simulink model "model"  (R2014a)
(part 2 of 2)

      | %<Vbase>V
      | %<VLF>pu
      | %<angleLF>deg.
      | %<Name>
  bus125 : powerlib/Measurements/Load Flow Bus  LConnTagsString=a  ID=bus125  Vbase=110000  Vref=1  Vangle=0  VLF=1  angleLF=0
      settings: AttributesFormatString=|
      | %<ID>
      | %<Vbase>V
      | %<VLF>pu
      | %<angleLF>deg.
      | %<Name>
  bus126 : powerlib/Measurements/Load Flow Bus  LConnTagsString=a  ID=bus126  Vbase=110000  Vref=1  Vangle=0  VLF=1  angleLF=0
      settings: AttributesFormatString=|
      | %<ID>
      | %<Vbase>V
      | %<VLF>pu
      | %<angleLF>deg.
      | %<Name>
  bus127 : powerlib/Measurements/Load Flow Bus  LConnTagsString=a  ID=bus127  Vbase=110000  Vref=1  Vangle=0  VLF=1  angleLF=0
      settings: AttributesFormatString=|
      | %<ID>
      | %<Vbase>V
      | %<VLF>pu
      | %<angleLF>deg.
      | %<Name>
  bus128 : powerlib/Measurements/Load Flow Bus  LConnTagsString=a  ID=bus128  Vbase=110000  Vref=1  Vangle=0  VLF=1  angleLF=0
      settings: AttributesFormatString=|
      | %<ID>
      | %<Vbase>V
      | %<VLF>pu
      | %<angleLF>deg.
      | %<Name>
  bus129 : powerlib/Measurements/Load Flow Bus  LConnTagsString=a  ID=bus129  Vbase=110000  Vref=1  Vangle=0  VLF=1  angleLF=0
      settings: AttributesFormatString=|
      | %<ID>
      | %<Vbase>V
      | %<VLF>pu
      | %<angleLF>deg.
      | %<Name>
  bus13 : powerlib/Measurements/Load Flow Bus  LConnTagsString=a  ID=bus13  Vbase=110000  Vref=1  Vangle=0  VLF=1  angleLF=0
      settings: AttributesFormatString=|
      | %<ID>
      | %<Vbase>V
      | %<VLF>pu
      | %<angleLF>deg.
      | %<Name>
  bus130 : powerlib/Measurements/Load Flow Bus  LConnTagsString=a  ID=bus130  Vbase=110000  Vref=1  Vangle=0  VLF=1  angleLF=0
      settings: AttributesFormatString=|
      | %<ID>
      | %<Vbase>V
      | %<VLF>pu
      | %<angleLF>deg.
      | %<Name>
  bus131 : powerlib/Measurements/Load Flow Bus  LConnTagsString=a  ID=bus131  Vbase=110000  Vref=1  Vangle=0  VLF=1  angleLF=0
      settings: AttributesFormatString=|
      | %<ID>
      | %<Vbase>V
      | %<VLF>pu
      | %<angleLF>deg.
      | %<Name>
  bus132 : powerlib/Measurements/Load Flow Bus  LConnTagsString=a  ID=bus132  Vbase=110000  Vref=1  Vangle=0  VLF=1  angleLF=0
      settings: AttributesFormatString=|
      | %<ID>
      | %<Vbase>V
      | %<VLF>pu
      | %<angleLF>deg.
      | %<Name>
  bus133 : powerlib/Measurements/Load Flow Bus  LConnTagsString=a  ID=bus133  Vbase=110000  Vref=1  Vangle=0  VLF=1  angleLF=0
      settings: AttributesFormatString=|
      | %<ID>
      | %<Vbase>V
      | %<VLF>pu
      | %<angleLF>deg.
      | %<Name>
  bus134 : powerlib/Measurements/Load Flow Bus  LConnTagsString=a  ID=bus134  Vbase=110000  Vref=1  Vangle=0  VLF=1  angleLF=0
      settings: AttributesFormatString=|
      | %<ID>
      | %<Vbase>V
      | %<VLF>pu
      | %<angleLF>deg.
      | %<Name>
  bus135 : powerlib/Measurements/Load Flow Bus  LConnTagsString=a  ID=bus135  Vbase=110000  Vref=1  Vangle=0  VLF=1  angleLF=0
      settings: AttributesFormatString=|
      | %<ID>
      | %<Vbase>V
      | %<VLF>pu
      | %<angleLF>deg.
      | %<Name>
  bus136 : powerlib/Measurements/Load Flow Bus  LConnTagsString=a  ID=bus136  Vbase=220000  Vref=1  Vangle=0  VLF=1  angleLF=0
      settings: AttributesFormatString=|
      | %<ID>
      | %<Vbase>V
      | %<VLF>pu
      | %<angleLF>deg.
      | %<Name>
  bus137 : powerlib/Measurements/Load Flow Bus  LConnTagsString=a  ID=bus137  Vbase=220000  Vref=1  Vangle=0  VLF=1  angleLF=0
      settings: AttributesFormatString=|
      | %<ID>
      | %<Vbase>V
      | %<VLF>pu
      | %<angleLF>deg.
      | %<Name>
  bus138 : powerlib/Measurements/Load Flow Bus  LConnTagsString=a  ID=bus138  Vbase=220000  Vref=1  Vangle=0  VLF=1  angleLF=0
      settings: AttributesFormatString=|
      | %<ID>
      | %<Vbase>V
      | %<VLF>pu
      | %<angleLF>deg.
      | %<Name>
  bus139 : powerlib/Measurements/Load Flow Bus  LConnTagsString=a  ID=bus139  Vbase=220000  Vref=1  Vangle=0  VLF=1  angleLF=0
      settings: AttributesFormatString=|
      | %<ID>
      | %<Vbase>V
      | %<VLF>pu
      | %<angleLF>deg.
      | %<Name>
  bus14 : powerlib/Measurements/Load Flow Bus  LConnTagsString=a  ID=bus14  Vbase=110000  Vref=1  Vangle=0  VLF=1  angleLF=0
      settings: AttributesFormatString=|
      | %<ID>
      | %<Vbase>V
      | %<VLF>pu
      | %<angleLF>deg.
      | %<Name>
  bus140 : powerlib/Measurements/Load Flow Bus  LConnTagsString=a  ID=bus140  Vbase=220000  Vref=1  Vangle=0  VLF=1  angleLF=0
      settings: AttributesFormatString=|
      | %<ID>
      | %<Vbase>V
      | %<VLF>pu
      | %<angleLF>deg.
      | %<Name>
  bus141 : powerlib/Measurements/Load Flow Bus  LConnTagsString=a  ID=bus141  Vbase=220000  Vref=1  Vangle=0  VLF=1  angleLF=0
      settings: AttributesFormatString=|
      | %<ID>
      | %<Vbase>V
      | %<VLF>pu
      | %<angleLF>deg.
      | %<Name>
  bus142 : powerlib/Measurements/Load Flow Bus  LConnTagsString=a  ID=bus142  Vbase=220000  Vref=1  Vangle=0  VLF=1  angleLF=0
      settings: AttributesFormatString=|
      | %<ID>
      | %<Vbase>V
      | %<VLF>pu
      | %<angleLF>deg.
      | %<Name>
  bus143 : powerlib/Measurements/Load Flow Bus  LConnTagsString=a  ID=bus143  Vbase=220000  Vref=1  Vangle=0  VLF=1  angleLF=0
      settings: AttributesFormatString=|
      | %<ID>
      | %<Vbase>V
      | %<VLF>pu
      | %<angleLF>deg.
      | %<Name>
  bus144 : powerlib/Measurements/Load Flow Bus  LConnTagsString=a  ID=bus144  Vbase=220000  Vref=1  Vangle=0  VLF=1  angleLF=0
      settings: AttributesFormatString=|
      | %<ID>
      | %<Vbase>V
      | %<VLF>pu
      | %<angleLF>deg.
      | %<Name>
  bus145 : powerlib/Measurements/Load Flow Bus  LConnTagsString=a  ID=bus145  Vbase=220000  Vref=1  Vangle=0  VLF=1  angleLF=0
      settings: AttributesFormatString=|
      | %<ID>
      | %<Vbase>V
      | %<VLF>pu
      | %<angleLF>deg.
      | %<Name>
  bus146 : powerlib/Measurements/Load Flow Bus  LConnTagsString=a  ID=bus146  Vbase=220000  Vref=1  Vangle=0  VLF=1  angleLF=0
      settings: AttributesFormatString=|
      | %<ID>
      | %<Vbase>V
      | %<VLF>pu
      | %<angleLF>deg.
      | %<Name>
  bus147 : powerlib/Measurements/Load Flow Bus  LConnTagsString=a  ID=bus147  Vbase=220000  Vref=1  Vangle=0  VLF=1  angleLF=0
      settings: AttributesFormatString=|
      | %<ID>
      | %<Vbase>V
      | %<VLF>pu
      | %<angleLF>deg.
      | %<Name>
  bus148 : powerlib/Measurements/Load Flow Bus  LConnTagsString=a  ID=bus148  Vbase=220000  Vref=1  Vangle=0  VLF=1  angleLF=0
      settings: AttributesFormatString=|
      | %<ID>
      | %<Vbase>V
      | %<VLF>pu
      | %<angleLF>deg.
      | %<Name>
  bus149 : powerlib/Measurements/Load Flow Bus  LConnTagsString=a  ID=bus149  Vbase=220000  Vref=1  Vangle=0  VLF=1  angleLF=0
      settings: AttributesFormatString=|
      | %<ID>
      | %<Vbase>V
      | %<VLF>pu
      | %<angleLF>deg.
      | %<Name>
  bus15 : powerlib/Measurements/Load Flow Bus  LConnTagsString=a  ID=bus15  Vbase=110000  Vref=1  Vangle=0  VLF=1  angleLF=0
      settings: AttributesFormatString=|
      | %<ID>
      | %<Vbase>V
      | %<VLF>pu
      | %<angleLF>deg.
      | %<Name>
  bus150 : powerlib/Measurements/Load Flow Bus  LConnTagsString=a  ID=bus150  Vbase=220000  Vref=1  Vangle=0  VLF=1  angleLF=0
      settings: AttributesFormatString=|
      | %<ID>
      | %<Vbase>V
      | %<VLF>pu
      | %<angleLF>deg.
      | %<Name>
  bus151 : powerlib/Measurements/Load Flow Bus  LConnTagsString=a  ID=bus151  Vbase=220000  Vref=1  Vangle=0  VLF=1  angleLF=0
      settings: AttributesFormatString=|
      | %<ID>
      | %<Vbase>V
      | %<VLF>pu
      | %<angleLF>deg.
      | %<Name>
  bus152 : powerlib/Measurements/Load Flow Bus  LConnTagsString=a  ID=bus152  Vbase=220000  Vref=1  Vangle=0  VLF=1  angleLF=0
      settings: AttributesFormatString=|
      | %<ID>
      | %<Vbase>V
      | %<VLF>pu
      | %<angleLF>deg.
      | %<Name>
  bus153 : powerlib/Measurements/Load Flow Bus  LConnTagsString=a  ID=bus153  Vbase=220000  Vref=1  Vangle=0  VLF=1  angleLF=0
      settings: AttributesFormatString=|
      | %<ID>
      | %<Vbase>V
      | %<VLF>pu
      | %<angleLF>deg.
      | %<Name>
  bus154 : powerlib/Measurements/Load Flow Bus  LConnTagsString=a  ID=bus154  Vbase=220000  Vref=1  Vangle=0  VLF=1  angleLF=0
      settings: AttributesFormatString=|
      | %<ID>
      | %<Vbase>V
      | %<VLF>pu
      | %<angleLF>deg.
      | %<Name>
  bus155 : powerlib/Measurements/Load Flow Bus  LConnTagsString=a  ID=bus155  Vbase=220000  Vref=1  Vangle=0  VLF=1  angleLF=0
      settings: AttributesFormatString=|
      | %<ID>
      | %<Vbase>V
      | %<VLF>pu
      | %<angleLF>deg.
      | %<Name>
  bus156 : powerlib/Measurements/Load Flow Bus  LConnTagsString=a  ID=bus156  Vbase=220000  Vref=1  Vangle=0  VLF=1  angleLF=0
      settings: AttributesFormatString=|
      | %<ID>
      | %<Vbase>V
      | %<VLF>pu
      | %<angleLF>deg.
      | %<Name>
  bus157 : powerlib/Measurements/Load Flow Bus  LConnTagsString=a  ID=bus157  Vbase=220000  Vref=1  Vangle=0  VLF=1  angleLF=0
      settings: AttributesFormatString=|
      | %<ID>
      | %<Vbase>V
      | %<VLF>pu
      | %<angleLF>deg.
      | %<Name>
  bus158 : powerlib/Measurements/Load Flow Bus  LConnTagsString=a  ID=bus158  Vbase=220000  Vref=1  Vangle=0  VLF=1  angleLF=0
      settings: AttributesFormatString=|
      | %<ID>
      | %<Vbase>V
      | %<VLF>pu
      | %<angleLF>deg.
      | %<Name>
  bus159 : powerlib/Measurements/Load Flow Bus  LConnTagsString=a  ID=bus159  Vbase=220000  Vref=1  Vangle=0  VLF=1  angleLF=0
      settings: AttributesFormatString=|
      | %<ID>
      | %<Vbase>V
      | %<VLF>pu
      | %<angleLF>deg.
      | %<Name>
  bus16 : powerlib/Measurements/Load Flow Bus  LConnTagsString=a  ID=bus16  Vbase=110000  Vref=1  Vangle=0  VLF=1  angleLF=0
      settings: AttributesFormatString=|
      | %<ID>
      | %<Vbase>V
      | %<VLF>pu
      | %<angleLF>deg.
      | %<Name>
  bus160 : powerlib/Measurements/Load Flow Bus  LConnTagsString=a  ID=bus160  Vbase=220000  Vref=1  Vangle=0  VLF=1  angleLF=0
      settings: AttributesFormatString=|
      | %<ID>
      | %<Vbase>V
      | %<VLF>pu
      | %<angleLF>deg.
      | %<Name>
  bus161 : powerlib/Measurements/Load Flow Bus  LConnTagsString=a  ID=bus161  Vbase=220000  Vref=1  Vangle=0  VLF=1  angleLF=0
      settings: AttributesFormatString=|
      | %<ID>
      | %<Vbase>V
      | %<VLF>pu
      | %<angleLF>deg.
      | %<Name>
  bus162 : powerlib/Measurements/Load Flow Bus  LConnTagsString=a  ID=bus162  Vbase=220000  Vref=1  Vangle=0  VLF=1  angleLF=0
      settings: AttributesFormatString=|
      | %<ID>
      | %<Vbase>V
      | %<VLF>pu
      | %<angleLF>deg.
      | %<Name>
  bus163 : powerlib/Measurements/Load Flow Bus  LConnTagsString=a  ID=bus163  Vbase=220000  Vref=1  Vangle=0  VLF=1  angleLF=0
      settings: AttributesFormatString=|
      | %<ID>
      | %<Vbase>V
      | %<VLF>pu
      | %<angleLF>deg.
      | %<Name>
  bus164 : powerlib/Measurements/Load Flow Bus  LConnTagsString=a  ID=bus164  Vbase=220000  Vref=1  Vangle=0  VLF=1  angleLF=0
      settings: AttributesFormatString=|
      | %<ID>
      | %<Vbase>V
      | %<VLF>pu
      | %<angleLF>deg.
      | %<Name>
  bus165 : powerlib/Measurements/Load Flow Bus  LConnTagsString=a  ID=bus165  Vbase=220000  Vref=1  Vangle=0  VLF=1  angleLF=0
      settings: AttributesFormatString=|
      | %<ID>
      | %<Vbase>V
      | %<VLF>pu
      | %<angleLF>deg.
      | %<Name>
  bus166 : powerlib/Measurements/Load Flow Bus  LConnTagsString=a  ID=bus166  Vbase=220000  Vref=1  Vangle=0  VLF=1  angleLF=0
      settings: AttributesFormatString=|
      | %<ID>
      | %<Vbase>V
      | %<VLF>pu
      | %<angleLF>deg.
      | %<Name>
  bus167 : powerlib/Measurements/Load Flow Bus  LConnTagsString=a  ID=bus167  Vbase=220000  Vref=1  Vangle=0  VLF=1  angleLF=0
      settings: AttributesFormatString=|
      | %<ID>
      | %<Vbase>V
      | %<VLF>pu
      | %<angleLF>deg.
      | %<Name>
  bus168 : powerlib/Measurements/Load Flow Bus  LConnTagsString=a  ID=bus168  Vbase=220000  Vref=1  Vangle=0  VLF=1  angleLF=0
      settings: AttributesFormatString=|
      | %<ID>
      | %<Vbase>V
      | %<VLF>pu
      | %<angleLF>deg.
      | %<Name>
  bus169 : powerlib/Measurements/Load Flow Bus  LConnTagsString=a  ID=bus169  Vbase=220000  Vref=1  Vangle=0  VLF=1  angleLF=0
      settings: AttributesFormatString=|
      | %<ID>
      | %<Vbase>V
      | %<VLF>pu
      | %<angleLF>deg.
      | %<Name>
  bus17 : powerlib/Measurements/Load Flow Bus  LConnTagsString=a  ID=bus17  Vbase=110000  Vref=1  Vangle=0  VLF=1  angleLF=0
      settings: AttributesFormatString=|
      | %<ID>
      | %<Vbase>V
      | %<VLF>pu
      | %<angleLF>deg.
      | %<Name>
  bus170 : powerlib/Measurements/Load Flow Bus  LConnTagsString=a  ID=bus170  Vbase=220000  Vref=1  Vangle=0  VLF=1  angleLF=0
      settings: AttributesFormatString=|
      | %<ID>
      | %<Vbase>V
      | %<VLF>pu
      | %<angleLF>deg.
      | %<Name>
  bus171 : powerlib/Measurements/Load Flow Bus  LConnTagsString=a  ID=bus171  Vbase=220000  Vref=1  Vangle=0  VLF=1  angleLF=0
      settings: AttributesFormatString=|
      | %<ID>
      | %<Vbase>V
      | %<VLF>pu
      | %<angleLF>deg.
      | %<Name>
  bus172 : powerlib/Measurements/Load Flow Bus  LConnTagsString=a  ID=bus172  Vbase=220000  Vref=1  Vangle=0  VLF=1  angleLF=0
      settings: AttributesFormatString=|
      | %<ID>
      | %<Vbase>V
      | %<VLF>pu
      | %<angleLF>deg.
      | %<Name>
  bus173 : powerlib/Measurements/Load Flow Bus  LConnTagsString=a  ID=bus173  Vbase=220000  Vref=1  Vangle=0  VLF=1  angleLF=0
      settings: AttributesFormatString=|
      | %<ID>
      | %<Vbase>V
      | %<VLF>pu
      | %<angleLF>deg.
      | %<Name>
  bus174 : powerlib/Measurements/Load Flow Bus  LConnTagsString=a  ID=bus174  Vbase=220000  Vref=1  Vangle=0  VLF=1  angleLF=0
      settings: AttributesFormatString=|
      | %<ID>
      | %<Vbase>V
      | %<VLF>pu
      | %<angleLF>deg.
      | %<Name>
  bus175 : powerlib/Measurements/Load Flow Bus  LConnTagsString=a  ID=bus175  Vbase=220000  Vref=1  Vangle=0  VLF=1  angleLF=0
      settings: AttributesFormatString=|
      | %<ID>
      | %<Vbase>V
      | %<VLF>pu
      | %<angleLF>deg.
      | %<Name>
  bus176 : powerlib/Measurements/Load Flow Bus  LConnTagsString=a  ID=bus176  Vbase=220000  Vref=1  Vangle=0  VLF=1  angleLF=0
      settings: AttributesFormatString=|
      | %<ID>
      | %<Vbase>V
      | %<VLF>pu
      | %<angleLF>deg.
      | %<Name>
  bus177 : powerlib/Measurements/Load Flow Bus  LConnTagsString=a  ID=bus177  Vbase=220000  Vref=1  Vangle=0  VLF=1  angleLF=0
      settings: AttributesFormatString=|
      | %<ID>
      | %<Vbase>V
      | %<VLF>pu
      | %<angleLF>deg.
      | %<Name>
  bus178 : powerlib/Measurements/Load Flow Bus  LConnTagsString=a  ID=bus178  Vbase=220000  Vref=1  Vangle=0  VLF=1  angleLF=0
      settings: AttributesFormatString=|
      | %<ID>
      | %<Vbase>V
      | %<VLF>pu
      | %<angleLF>deg.
      | %<Name>
  bus179 : powerlib/Measurements/Load Flow Bus  LConnTagsString=a  ID=bus179  Vbase=220000  Vref=1  Vangle=0  VLF=1  angleLF=0
      settings: AttributesFormatString=|
      | %<ID>
      | %<Vbase>V
      | %<VLF>pu
      | %<angleLF>deg.
      | %<Name>
  bus18 : powerlib/Measurements/Load Flow Bus  LConnTagsString=a  ID=bus18  Vbase=110000  Vref=1  Vangle=0  VLF=1  angleLF=0
      settings: AttributesFormatString=|
      | %<ID>
      | %<Vbase>V
      | %<VLF>pu
      | %<angleLF>deg.
      | %<Name>
  bus180 : powerlib/Measurements/Load Flow Bus  LConnTagsString=a  ID=bus180  Vbase=220000  Vref=1  Vangle=0  VLF=1  angleLF=0
      settings: AttributesFormatString=|
      | %<ID>
      | %<Vbase>V
      | %<VLF>pu
      | %<angleLF>deg.
      | %<Name>
  bus181 : powerlib/Measurements/Load Flow Bus  LConnTagsString=a  ID=bus181  Vbase=220000  Vref=1  Vangle=0  VLF=1  angleLF=0
      settings: AttributesFormatString=|
      | %<ID>
      | %<Vbase>V
      | %<VLF>pu
      | %<angleLF>deg.
      | %<Name>
  bus182 : powerlib/Measurements/Load Flow Bus  LConnTagsString=a  ID=bus182  Vbase=220000  Vref=1  Vangle=0  VLF=1  angleLF=0
      settings: AttributesFormatString=|
      | %<ID>
      | %<Vbase>V
      | %<VLF>pu
      | %<angleLF>deg.
      | %<Name>
  bus183 : powerlib/Measurements/Load Flow Bus  LConnTagsString=a  ID=bus183  Vbase=220000  Vref=1  Vangle=0  VLF=1  angleLF=0
      settings: AttributesFormatString=|
      | %<ID>
      | %<Vbase>V
      | %<VLF>pu
      | %<angleLF>deg.
      | %<Name>
  bus184 : powerlib/Measurements/Load Flow Bus  LConnTagsString=a  ID=bus184  Vbase=220000  Vref=1  Vangle=0  VLF=1  angleLF=0
      settings: AttributesFormatString=|
      | %<ID>
      | %<Vbase>V
      | %<VLF>pu
      | %<angleLF>deg.
      | %<Name>
  bus185 : powerlib/Measurements/Load Flow Bus  LConnTagsString=a  ID=bus185  Vbase=220000  Vref=1  Vangle=0  VLF=1  angleLF=0
      settings: AttributesFormatString=|
      | %<ID>
      | %<Vbase>V
      | %<VLF>pu
      | %<angleLF>deg.
      | %<Name>
  bus186 : powerlib/Measurements/Load Flow Bus  LConnTagsString=a  ID=bus186  Vbase=220000  Vref=1  Vangle=0  VLF=1  angleLF=0
      settings: AttributesFormatString=|
      | %<ID>
      | %<Vbase>V
      | %<VLF>pu
      | %<angleLF>deg.
      | %<Name>
  bus187 : powerlib/Measurements/Load Flow Bus  LConnTagsString=a  ID=bus187  Vbase=220000  Vref=1  Vangle=0  VLF=1  angleLF=0
      settings: AttributesFormatString=|
      | %<ID>
      | %<Vbase>V
      | %<VLF>pu
      | %<angleLF>deg.
      | %<Name>
  bus188 : powerlib/Measurements/Load Flow Bus  LConnTagsString=a  ID=bus188  Vbase=220000  Vref=1  Vangle=0  VLF=1  angleLF=0
      settings: AttributesFormatString=|
      | %<ID>
      | %<Vbase>V
      | %<VLF>pu
      | %<angleLF>deg.
      | %<Name>
  bus189 : powerlib/Measurements/Load Flow Bus  LConnTagsString=a  ID=bus189  Vbase=220000  Vref=1  Vangle=0  VLF=1  angleLF=0
      settings: AttributesFormatString=|
      | %<ID>
      | %<Vbase>V
      | %<VLF>pu
      | %<angleLF>deg.
      | %<Name>
  bus19 : powerlib/Measurements/Load Flow Bus  LConnTagsString=a  ID=bus19  Vbase=110000  Vref=1  Vangle=0  VLF=1  angleLF=0
      settings: AttributesFormatString=|
      | %<ID>
      | %<Vbase>V
      | %<VLF>pu
      | %<angleLF>deg.
      | %<Name>
  bus190 : powerlib/Measurements/Load Flow Bus  LConnTagsString=a  ID=bus190  Vbase=220000  Vref=1  Vangle=0  VLF=1  angleLF=0
      settings: AttributesFormatString=|
      | %<ID>
      | %<Vbase>V
      | %<VLF>pu
      | %<angleLF>deg.
      | %<Name>
  bus191 : powerlib/Measurements/Load Flow Bus  LConnTagsString=a  ID=bus191  Vbase=220000  Vref=1  Vangle=0  VLF=1  angleLF=0
      settings: AttributesFormatString=|
      | %<ID>
      | %<Vbase>V
      | %<VLF>pu
      | %<angleLF>deg.
      | %<Name>
  bus192 : powerlib/Measurements/Load Flow Bus  LConnTagsString=a  ID=bus192  Vbase=220000  Vref=1  Vangle=0  VLF=1  angleLF=0
      settings: AttributesFormatString=|
      | %<ID>
      | %<Vbase>V
      | %<VLF>pu
      | %<angleLF>deg.
      | %<Name>
  bus193 : powerlib/Measurements/Load Flow Bus  LConnTagsString=a  ID=bus193  Vbase=220000  Vref=1  Vangle=0  VLF=1  angleLF=0
      settings: AttributesFormatString=|
      | %<ID>
      | %<Vbase>V
      | %<VLF>pu
      | %<angleLF>deg.
      | %<Name>
  bus194 : powerlib/Measurements/Load Flow Bus  LConnTagsString=a  ID=bus194  Vbase=220000  Vref=1  Vangle=0  VLF=1  angleLF=0
      settings: AttributesFormatString=|
      | %<ID>
      | %<Vbase>V
      | %<VLF>pu
      | %<angleLF>deg.
      | %<Name>
  bus195 : powerlib/Measurements/Load Flow Bus  LConnTagsString=a  ID=bus195  Vbase=220000  Vref=1  Vangle=0  VLF=1  angleLF=0
      settings: AttributesFormatString=|
      | %<ID>
      | %<Vbase>V
      | %<VLF>pu
      | %<angleLF>deg.
      | %<Name>
  bus196 : powerlib/Measurements/Load Flow Bus  LConnTagsString=a  ID=bus196  Vbase=220000  Vref=1  Vangle=0  VLF=1  angleLF=0
      settings: AttributesFormatString=|
      | %<ID>
      | %<Vbase>V
      | %<VLF>pu
      | %<angleLF>deg.
      | %<Name>
  bus197 : powerlib/Measurements/Load Flow Bus  LConnTagsString=a  ID=bus197  Vbase=220000  Vref=1  Vangle=0  VLF=1  angleLF=0
      settings: AttributesFormatString=|
      | %<ID>
      | %<Vbase>V
      | %<VLF>pu
      | %<angleLF>deg.
      | %<Name>
  bus198 : powerlib/Measurements/Load Flow Bus  LConnTagsString=a  ID=bus198  Vbase=220000  Vref=1  Vangle=0  VLF=1  angleLF=0
      settings: AttributesFormatString=|
      | %<ID>
      | %<Vbase>V
      | %<VLF>pu
      | %<angleLF>deg.
      | %<Name>
  bus199 : powerlib/Measurements/Load Flow Bus  LConnTagsString=a  ID=bus199  Vbase=220000  Vref=1  Vangle=0  VLF=1  angleLF=0
      settings: AttributesFormatString=|
      | %<ID>
      | %<Vbase>V
      | %<VLF>pu
      | %<angleLF>deg.
      | %<Name>
  bus2 : powerlib/Measurements/Load Flow Bus  LConnTagsString=a  ID=bus2  Vbase=110000  Vref=1  Vangle=0  VLF=1  angleLF=0
      settings: AttributesFormatString=|
      | %<ID>
      | %<Vbase>V
      | %<VLF>pu
      | %<angleLF>deg.
      | %<Name>
  bus20 : powerlib/Measurements/Load Flow Bus  LConnTagsString=a  ID=bus20  Vbase=110000  Vref=1  Vangle=0  VLF=1  angleLF=0
      settings: AttributesFormatString=|
      | %<ID>
      | %<Vbase>V
      | %<VLF>pu
      | %<angleLF>deg.
      | %<Name>
  bus200 : powerlib/Measurements/Load Flow Bus  LConnTagsString=a  ID=bus200  Vbase=220000  Vref=1  Vangle=0  VLF=1  angleLF=0
      settings: AttributesFormatString=|
      | %<ID>
      | %<Vbase>V
      | %<VLF>pu
      | %<angleLF>deg.
      | %<Name>
  bus201 : powerlib/Measurements/Load Flow Bus  LConnTagsString=a  ID=bus201  Vbase=220000  Vref=1  Vangle=0  VLF=1  angleLF=0
      settings: AttributesFormatString=|
      | %<ID>
      | %<Vbase>V
      | %<VLF>pu
      | %<angleLF>deg.
      | %<Name>
  bus202 : powerlib/Measurements/Load Flow Bus  LConnTagsString=a  ID=bus202  Vbase=220000  Vref=1  Vangle=0  VLF=1  angleLF=0
      settings: AttributesFormatString=|
      | %<ID>
      | %<Vbase>V
      | %<VLF>pu
      | %<angleLF>deg.
      | %<Name>
  bus203 : powerlib/Measurements/Load Flow Bus  LConnTagsString=a  ID=bus203  Vbase=220000  Vref=1  Vangle=0  VLF=1  angleLF=0
      settings: AttributesFormatString=|
      | %<ID>
      | %<Vbase>V
      | %<VLF>pu
      | %<angleLF>deg.
      | %<Name>
  bus204 : powerlib/Measurements/Load Flow Bus  LConnTagsString=a  ID=bus204  Vbase=220000  Vref=1  Vangle=0  VLF=1  angleLF=0
      settings: AttributesFormatString=|
      | %<ID>
      | %<Vbase>V
      | %<VLF>pu
      | %<angleLF>deg.
      | %<Name>
  bus205 : powerlib/Measurements/Load Flow Bus  LConnTagsString=a  ID=bus205  Vbase=220000  Vref=1  Vangle=0  VLF=1  angleLF=0
      settings: AttributesFormatString=|
      | %<ID>
      | %<Vbase>V
      | %<VLF>pu
      | %<angleLF>deg.
      | %<Name>
  bus206 : powerlib/Measurements/Load Flow Bus  LConnTagsString=a  ID=bus206  Vbase=220000  Vref=1  Vangle=0  VLF=1  angleLF=0
      settings: AttributesFormatString=|
      | %<ID>
      | %<Vbase>V
      | %<VLF>pu
      | %<angleLF>deg.
      | %<Name>
  bus207 : powerlib/Measurements/Load Flow Bus  LConnTagsString=a  ID=bus207  Vbase=220000  Vref=1  Vangle=0  VLF=1  angleLF=0
      settings: AttributesFormatString=|
      | %<ID>
      | %<Vbase>V
      | %<VLF>pu
      | %<angleLF>deg.
      | %<Name>
  bus208 : powerlib/Measurements/Load Flow Bus  LConnTagsString=a  ID=bus208  Vbase=220000  Vref=1  Vangle=0  VLF=1  angleLF=0
      settings: AttributesFormatString=|
      | %<ID>
      | %<Vbase>V
      | %<VLF>pu
      | %<angleLF>deg.
      | %<Name>
  bus209 : powerlib/Measurements/Load Flow Bus  LConnTagsString=a  ID=bus209  Vbase=220000  Vref=1  Vangle=0  VLF=1  angleLF=0
      settings: AttributesFormatString=|
      | %<ID>
      | %<Vbase>V
      | %<VLF>pu
      | %<angleLF>deg.
      | %<Name>
  bus21 : powerlib/Measurements/Load Flow Bus  LConnTagsString=a  ID=bus21  Vbase=110000  Vref=1  Vangle=0  VLF=1  angleLF=0
      settings: AttributesFormatString=|
      | %<ID>
      | %<Vbase>V
      | %<VLF>pu
      | %<angleLF>deg.
      | %<Name>
  bus210 : powerlib/Measurements/Load Flow Bus  LConnTagsString=a  ID=bus210  Vbase=220000  Vref=1  Vangle=0  VLF=1  angleLF=0
      settings: AttributesFormatString=|
      | %<ID>
      | %<Vbase>V
      | %<VLF>pu
      | %<angleLF>deg.
      | %<Name>
  bus211 : powerlib/Measurements/Load Flow Bus  LConnTagsString=a  ID=bus211  Vbase=220000  Vref=1  Vangle=0  VLF=1  angleLF=0
      settings: AttributesFormatString=|
      | %<ID>
      | %<Vbase>V
      | %<VLF>pu
      | %<angleLF>deg.
      | %<Name>
  bus212 : powerlib/Measurements/Load Flow Bus  LConnTagsString=a  ID=bus212  Vbase=220000  Vref=1  Vangle=0  VLF=1  angleLF=0
      settings: AttributesFormatString=|
      | %<ID>
      | %<Vbase>V
      | %<VLF>pu
      | %<angleLF>deg.
      | %<Name>
  bus213 : powerlib/Measurements/Load Flow Bus  LConnTagsString=a  ID=bus213  Vbase=220000  Vref=1  Vangle=0  VLF=1  angleLF=0
      settings: AttributesFormatString=|
      | %<ID>
      | %<Vbase>V
      | %<VLF>pu
      | %<angleLF>deg.
      | %<Name>
  bus214 : powerlib/Measurements/Load Flow Bus  LConnTagsString=a  ID=bus214  Vbase=220000  Vref=1  Vangle=0  VLF=1  angleLF=0
      settings: AttributesFormatString=|
      | %<ID>
      | %<Vbase>V
      | %<VLF>pu
      | %<angleLF>deg.
      | %<Name>
  bus215 : powerlib/Measurements/Load Flow Bus  LConnTagsString=a  ID=bus215  Vbase=220000  Vref=1  Vangle=0  VLF=1  angleLF=0
      settings: AttributesFormatString=|
      | %<ID>
      | %<Vbase>V
      | %<VLF>pu
      | %<angleLF>deg.
      | %<Name>
  bus216 : powerlib/Measurements/Load Flow Bus  LConnTagsString=a  ID=bus216  Vbase=220000  Vref=1  Vangle=0  VLF=1  angleLF=0
      settings: AttributesFormatString=|
      | %<ID>
      | %<Vbase>V
      | %<VLF>pu
      | %<angleLF>deg.
      | %<Name>
  bus217 : powerlib/Measurements/Load Flow Bus  LConnTagsString=a  ID=bus217  Vbase=220000  Vref=1  Vangle=0  VLF=1  angleLF=0
      settings: AttributesFormatString=|
      | %<ID>
      | %<Vbase>V
      | %<VLF>pu
      | %<angleLF>deg.
      | %<Name>
  bus218 : powerlib/Measurements/Load Flow Bus  LConnTagsString=a  ID=bus218  Vbase=220000  Vref=1  Vangle=0  VLF=1  angleLF=0
      settings: AttributesFormatString=|
      | %<ID>
      | %<Vbase>V
      | %<VLF>pu
      | %<angleLF>deg.
      | %<Name>
  bus219 : powerlib/Measurements/Load Flow Bus  LConnTagsString=a  ID=bus219  Vbase=220000  Vref=1  Vangle=0  VLF=1  angleLF=0
      settings: AttributesFormatString=|
      | %<ID>
      | %<Vbase>V
      | %<VLF>pu
      | %<angleLF>deg.
      | %<Name>
  bus22 : powerlib/Measurements/Load Flow Bus  LConnTagsString=a  ID=bus22  Vbase=110000  Vref=1  Vangle=0  VLF=1  angleLF=0
      settings: AttributesFormatString=|
      | %<ID>
      | %<Vbase>V
      | %<VLF>pu
      | %<angleLF>deg.
      | %<Name>
  bus220 : powerlib/Measurements/Load Flow Bus  LConnTagsString=a  ID=bus220  Vbase=220000  Vref=1  Vangle=0  VLF=1  angleLF=0
      settings: AttributesFormatString=|
      | %<ID>
      | %<Vbase>V
      | %<VLF>pu
      | %<angleLF>deg.
      | %<Name>
  bus221 : powerlib/Measurements/Load Flow Bus  LConnTagsString=a  ID=bus221  Vbase=220000  Vref=1  Vangle=0  VLF=1  angleLF=0
      settings: AttributesFormatString=|
      | %<ID>
      | %<Vbase>V
      | %<VLF>pu
      | %<angleLF>deg.
      | %<Name>
  bus222 : powerlib/Measurements/Load Flow Bus  LConnTagsString=a  ID=bus222  Vbase=220000  Vref=1  Vangle=0  VLF=1  angleLF=0
      settings: AttributesFormatString=|
      | %<ID>
      | %<Vbase>V
      | %<VLF>pu
      | %<angleLF>deg.
      | %<Name>
  bus23 : powerlib/Measurements/Load Flow Bus  LConnTagsString=a  ID=bus23  Vbase=110000  Vref=1  Vangle=0  VLF=1  angleLF=0
      settings: AttributesFormatString=|
      | %<ID>
      | %<Vbase>V
      | %<VLF>pu
      | %<angleLF>deg.
      | %<Name>
  bus24 : powerlib/Measurements/Load Flow Bus  LConnTagsString=a  ID=bus24  Vbase=110000  Vref=1  Vangle=0  VLF=1  angleLF=0
      settings: AttributesFormatString=|
      | %<ID>
      | %<Vbase>V
      | %<VLF>pu
      | %<angleLF>deg.
      | %<Name>
  bus25 : powerlib/Measurements/Load Flow Bus  LConnTagsString=a  ID=bus25  Vbase=220000  Vref=1  Vangle=0  VLF=1  angleLF=0
      settings: AttributesFormatString=|
      | %<ID>
      | %<Vbase>V
      | %<VLF>pu
      | %<angleLF>deg.
      | %<Name>
  bus26 : powerlib/Measurements/Load Flow Bus  LConnTagsString=a  ID=bus26  Vbase=220000  Vref=1  Vangle=0  VLF=1  angleLF=0
      settings: AttributesFormatString=|
      | %<ID>
      | %<Vbase>V
      | %<VLF>pu
      | %<angleLF>deg.
      | %<Name>
  bus27 : powerlib/Measurements/Load Flow Bus  LConnTagsString=a  ID=bus27  Vbase=220000  Vref=1  Vangle=0  VLF=1  angleLF=0
      settings: AttributesFormatString=|
      | %<ID>
      | %<Vbase>V
      | %<VLF>pu
      | %<angleLF>deg.
      | %<Name>
  bus28 : powerlib/Measurements/Load Flow Bus  LConnTagsString=a  ID=bus28  Vbase=220000  Vref=1  Vangle=0  VLF=1  angleLF=0
      settings: AttributesFormatString=|
      | %<ID>
      | %<Vbase>V
      | %<VLF>pu
      | %<angleLF>deg.
      | %<Name>
  bus29 : powerlib/Measurements/Load Flow Bus  LConnTagsString=a  ID=bus29  Vbase=220000  Vref=1  Vangle=0  VLF=1  angleLF=0
      settings: AttributesFormatString=|
      | %<ID>
      | %<Vbase>V
      | %<VLF>pu
      | %<angleLF>deg.
      | %<Name>
  bus3 : powerlib/Measurements/Load Flow Bus  LConnTagsString=a  ID=bus3  Vbase=110000  Vref=1  Vangle=0  VLF=1  angleLF=0
      settings: AttributesFormatString=|
      | %<ID>
      | %<Vbase>V
      | %<VLF>pu
      | %<angleLF>deg.
      | %<Name>
  bus30 : powerlib/Measurements/Load Flow Bus  LConnTagsString=a  ID=bus30  Vbase=220000  Vref=1  Vangle=0  VLF=1  angleLF=0
      settings: AttributesFormatString=|
      | %<ID>
      | %<Vbase>V
      | %<VLF>pu
      | %<angleLF>deg.
      | %<Name>
  bus31 : powerlib/Measurements/Load Flow Bus  LConnTagsString=a  ID=bus31  Vbase=220000  Vref=1  Vangle=0  VLF=1  angleLF=0
      settings: AttributesFormatString=|
      | %<ID>
      | %<Vbase>V
      | %<VLF>pu
      | %<angleLF>deg.
      | %<Name>
  bus32 : powerlib/Measurements/Load Flow Bus  LConnTagsString=a  ID=bus32  Vbase=220000  Vref=1  Vangle=0  VLF=1  angleLF=0
      settings: AttributesFormatString=|
      | %<ID>
      | %<Vbase>V
      | %<VLF>pu
      | %<angleLF>deg.
      | %<Name>
  bus33 : powerlib/Measurements/Load Flow Bus  LConnTagsString=a  ID=bus33  Vbase=220000  Vref=1  Vangle=0  VLF=1  angleLF=0
      settings: AttributesFormatString=|
      | %<ID>
      | %<Vbase>V
      | %<VLF>pu
      | %<angleLF>deg.
      | %<Name>
  bus34 : powerlib/Measurements/Load Flow Bus  LConnTagsString=a  ID=bus34  Vbase=220000  Vref=1  Vangle=0  VLF=1  angleLF=0
      settings: AttributesFormatString=|
      | %<ID>
      | %<Vbase>V
      | %<VLF>pu
      | %<angleLF>deg.
      | %<Name>
  bus35 : powerlib/Measurements/Load Flow Bus  LConnTagsString=a  ID=bus35  Vbase=220000  Vref=1  Vangle=0  VLF=1  angleLF=0
      settings: AttributesFormatString=|
      | %<ID>
      | %<Vbase>V
      | %<VLF>pu
      | %<angleLF>deg.
      | %<Name>
  bus36 : powerlib/Measurements/Load Flow Bus  LConnTagsString=a  ID=bus36  Vbase=220000  Vref=1  Vangle=0  VLF=1  angleLF=0
      settings: AttributesFormatString=|
      | %<ID>
      | %<Vbase>V
      | %<VLF>pu
      | %<angleLF>deg.
      | %<Name>
  bus37 : powerlib/Measurements/Load Flow Bus  LConnTagsString=a  ID=bus37  Vbase=220000  Vref=1  Vangle=0  VLF=1  angleLF=0
      settings: AttributesFormatString=|
      | %<ID>
      | %<Vbase>V
      | %<VLF>pu
      | %<angleLF>deg.
      | %<Name>
  bus38 : powerlib/Measurements/Load Flow Bus  LConnTagsString=a  ID=bus38  Vbase=220000  Vref=1  Vangle=0  VLF=1  angleLF=0
      settings: AttributesFormatString=|
      | %<ID>
      | %<Vbase>V
      | %<VLF>pu
      | %<angleLF>deg.
      | %<Name>
  bus39 : powerlib/Measurements/Load Flow Bus  LConnTagsString=a  ID=bus39  Vbase=220000  Vref=1  Vangle=0  VLF=1  angleLF=0
      settings: AttributesFormatString=|
      | %<ID>
      | %<Vbase>V
      | %<VLF>pu
      | %<angleLF>deg.
      | %<Name>
  bus4 : powerlib/Measurements/Load Flow Bus  LConnTagsString=a  ID=bus4  Vbase=110000  Vref=1  Vangle=0  VLF=1  angleLF=0
      settings: AttributesFormatString=|
      | %<ID>
      | %<Vbase>V
      | %<VLF>pu
      | %<angleLF>deg.
      | %<Name>
  bus40 : powerlib/Measurements/Load Flow Bus  LConnTagsString=a  ID=bus40  Vbase=220000  Vref=1  Vangle=0  VLF=1  angleLF=0
      settings: AttributesFormatString=|
      | %<ID>
      | %<Vbase>V
      | %<VLF>pu
      | %<angleLF>deg.
      | %<Name>
  bus41 : powerlib/Measurements/Load Flow Bus  LConnTagsString=a  ID=bus41  Vbase=220000  Vref=1  Vangle=0  VLF=1  angleLF=0
      settings: AttributesFormatString=|
      | %<ID>
      | %<Vbase>V
      | %<VLF>pu
      | %<angleLF>deg.
      | %<Name>
  bus42 : powerlib/Measurements/Load Flow Bus  LConnTagsString=a  ID=bus42  Vbase=220000  Vref=1  Vangle=0  VLF=1  angleLF=0
      settings: AttributesFormatString=|
      | %<ID>
      | %<Vbase>V
      | %<VLF>pu
      | %<angleLF>deg.
      | %<Name>
  bus43 : powerlib/Measurements/Load Flow Bus  LConnTagsString=a  ID=bus43  Vbase=220000  Vref=1  Vangle=0  VLF=1  angleLF=0
      settings: AttributesFormatString=|
      | %<ID>
      | %<Vbase>V
      | %<VLF>pu
      | %<angleLF>deg.
      | %<Name>
  bus44 : powerlib/Measurements/Load Flow Bus  LConnTagsString=a  ID=bus44  Vbase=220000  Vref=1  Vangle=0  VLF=1  angleLF=0
      settings: AttributesFormatString=|
      | %<ID>
      | %<Vbase>V
      | %<VLF>pu
      | %<angleLF>deg.
      | %<Name>
  bus45 : powerlib/Measurements/Load Flow Bus  LConnTagsString=a  ID=bus45  Vbase=220000  Vref=1  Vangle=0  VLF=1  angleLF=0
      settings: AttributesFormatString=|
      | %<ID>
      | %<Vbase>V
      | %<VLF>pu
      | %<angleLF>deg.
      | %<Name>
  bus46 : powerlib/Measurements/Load Flow Bus  LConnTagsString=a  ID=bus46  Vbase=220000  Vref=1  Vangle=0  VLF=1  angleLF=0
      settings: AttributesFormatString=|
      | %<ID>
      | %<Vbase>V
      | %<VLF>pu
      | %<angleLF>deg.
      | %<Name>
  bus47 : powerlib/Measurements/Load Flow Bus  LConnTagsString=a  ID=bus47  Vbase=220000  Vref=1  Vangle=0  VLF=1  angleLF=0
      settings: AttributesFormatString=|
      | %<ID>
      | %<Vbase>V
      | %<VLF>pu
      | %<angleLF>deg.
      | %<Name>
  bus48 : powerlib/Measurements/Load Flow Bus  LConnTagsString=a  ID=bus48  Vbase=220000  Vref=1  Vangle=0  VLF=1  angleLF=0
      settings: AttributesFormatString=|
      | %<ID>
      | %<Vbase>V
      | %<VLF>pu
      | %<angleLF>deg.
      | %<Name>
  bus49 : powerlib/Measurements/Load Flow Bus  LConnTagsString=a  ID=bus49  Vbase=220000  Vref=1  Vangle=0  VLF=1  angleLF=0
      settings: AttributesFormatString=|
      | %<ID>
      | %<Vbase>V
      | %<VLF>pu
      | %<angleLF>deg.
      | %<Name>
  bus5 : powerlib/Measurements/Load Flow Bus  LConnTagsString=a  ID=bus5  Vbase=110000  Vref=1  Vangle=0  VLF=1  angleLF=0
      settings: AttributesFormatString=|
      | %<ID>
      | %<Vbase>V
      | %<VLF>pu
      | %<angleLF>deg.
      | %<Name>
  bus50 : powerlib/Measurements/Load Flow Bus  LConnTagsString=a  ID=bus50  Vbase=220000  Vref=1  Vangle=0  VLF=1  angleLF=0
      settings: AttributesFormatString=|
      | %<ID>
      | %<Vbase>V
      | %<VLF>pu
      | %<angleLF>deg.
      | %<Name>
  bus51 : powerlib/Measurements/Load Flow Bus  LConnTagsString=a  ID=bus51  Vbase=220000  Vref=1  Vangle=0  VLF=1  angleLF=0
      settings: AttributesFormatString=|
      | %<ID>
      | %<Vbase>V
      | %<VLF>pu
      | %<angleLF>deg.
      | %<Name>
  bus52 : powerlib/Measurements/Load Flow Bus  LConnTagsString=a  ID=bus52  Vbase=220000  Vref=1  Vangle=0  VLF=1  angleLF=0
      settings: AttributesFormatString=|
      | %<ID>
      | %<Vbase>V
      | %<VLF>pu
      | %<angleLF>deg.
      | %<Name>
  bus53 : powerlib/Measurements/Load Flow Bus  LConnTagsString=a  ID=bus53  Vbase=220000  Vref=1  Vangle=0  VLF=1  angleLF=0
      settings: AttributesFormatString=|
      | %<ID>
      | %<Vbase>V
      | %<VLF>pu
      | %<angleLF>deg.
      | %<Name>
  bus54 : powerlib/Measurements/Load Flow Bus  LConnTagsString=a  ID=bus54  Vbase=220000  Vref=1  Vangle=0  VLF=1  angleLF=0
      settings: AttributesFormatString=|
      | %<ID>
      | %<Vbase>V
      | %<VLF>pu
      | %<angleLF>deg.
      | %<Name>
  bus55 : powerlib/Measurements/Load Flow Bus  LConnTagsString=a  ID=bus55  Vbase=220000  Vref=1  Vangle=0  VLF=1  angleLF=0
      settings: AttributesFormatString=|
      | %<ID>
      | %<Vbase>V
      | %<VLF>pu
      | %<angleLF>deg.
      | %<Name>
  bus56 : powerlib/Measurements/Load Flow Bus  LConnTagsString=a  ID=bus56  Vbase=220000  Vref=1  Vangle=0  VLF=1  angleLF=0
      settings: AttributesFormatString=|
      | %<ID>
      | %<Vbase>V
      | %<VLF>pu
      | %<angleLF>deg.
      | %<Name>
  bus57 : powerlib/Measurements/Load Flow Bus  LConnTagsString=a  ID=bus57  Vbase=220000  Vref=1  Vangle=0  VLF=1  angleLF=0
      settings: AttributesFormatString=|
      | %<ID>
      | %<Vbase>V
      | %<VLF>pu
      | %<angleLF>deg.
      | %<Name>
  bus58 : powerlib/Measurements/Load Flow Bus  LConnTagsString=a  ID=bus58  Vbase=220000  Vref=1  Vangle=0  VLF=1  angleLF=0
      settings: AttributesFormatString=|
      | %<ID>
      | %<Vbase>V
      | %<VLF>pu
      | %<angleLF>deg.
      | %<Name>
  bus59 : powerlib/Measurements/Load Flow Bus  LConnTagsString=a  ID=bus59  Vbase=220000  Vref=1  Vangle=0  VLF=1  angleLF=0
      settings: AttributesFormatString=|
      | %<ID>
      | %<Vbase>V
      | %<VLF>pu
      | %<angleLF>deg.
      | %<Name>
  bus6 : powerlib/Measurements/Load Flow Bus  LConnTagsString=a  ID=bus6  Vbase=110000  Vref=1  Vangle=0  VLF=1  angleLF=0
      settings: AttributesFormatString=|
      | %<ID>
      | %<Vbase>V
      | %<VLF>pu
      | %<angleLF>deg.
      | %<Name>
  bus60 : powerlib/Measurements/Load Flow Bus  LConnTagsString=a  ID=bus60  Vbase=220000  Vref=1  Vangle=0  VLF=1  angleLF=0
      settings: AttributesFormatString=|
      | %<ID>
      | %<Vbase>V
      | %<VLF>pu
      | %<angleLF>deg.
      | %<Name>
  bus61 : powerlib/Measurements/Load Flow Bus  LConnTagsString=a  ID=bus61  Vbase=220000  Vref=1  Vangle=0  VLF=1  angleLF=0
      settings: AttributesFormatString=|
      | %<ID>
      | %<Vbase>V
      | %<VLF>pu
      | %<angleLF>deg.
      | %<Name>
  bus62 : powerlib/Measurements/Load Flow Bus  LConnTagsString=a  ID=bus62  Vbase=220000  Vref=1  Vangle=0  VLF=1  angleLF=0
      settings: AttributesFormatString=|
      | %<ID>
      | %<Vbase>V
      | %<VLF>pu
      | %<angleLF>deg.
      | %<Name>
  bus63 : powerlib/Measurements/Load Flow Bus  LConnTagsString=a  ID=bus63  Vbase=220000  Vref=1  Vangle=0  VLF=1  angleLF=0
      settings: AttributesFormatString=|
      | %<ID>
      | %<Vbase>V
      | %<VLF>pu
      | %<angleLF>deg.
      | %<Name>
  bus64 : powerlib/Measurements/Load Flow Bus  LConnTagsString=a  ID=bus64  Vbase=220000  Vref=1  Vangle=0  VLF=1  angleLF=0
      settings: AttributesFormatString=|
      | %<ID>
      | %<Vbase>V
      | %<VLF>pu
      | %<angleLF>deg.
      | %<Name>
  bus65 : powerlib/Measurements/Load Flow Bus  LConnTagsString=a  ID=bus65  Vbase=220000  Vref=1  Vangle=0  VLF=1  angleLF=0
      settings: AttributesFormatString=|
      | %<ID>
      | %<Vbase>V
      | %<VLF>pu
      | %<angleLF>deg.
      | %<Name>
  bus66 : powerlib/Measurements/Load Flow Bus  LConnTagsString=a  ID=bus66  Vbase=220000  Vref=1  Vangle=0  VLF=1  angleLF=0
      settings: AttributesFormatString=|
      | %<ID>
      | %<Vbase>V
      | %<VLF>pu
      | %<angleLF>deg.
      | %<Name>
  bus67 : powerlib/Measurements/Load Flow Bus  LConnTagsString=a  ID=bus67  Vbase=220000  Vref=1  Vangle=0  VLF=1  angleLF=0
      settings: AttributesFormatString=|
      | %<ID>
      | %<Vbase>V
      | %<VLF>pu
      | %<angleLF>deg.
      | %<Name>
  bus68 : powerlib/Measurements/Load Flow Bus  LConnTagsString=a  ID=bus68  Vbase=220000  Vref=1  Vangle=0  VLF=1  angleLF=0
      settings: AttributesFormatString=|
      | %<ID>
      | %<Vbase>V
      | %<VLF>pu
      | %<angleLF>deg.
      | %<Name>
  bus69 : powerlib/Measurements/Load Flow Bus  LConnTagsString=a  ID=bus69  Vbase=220000  Vref=1  Vangle=0  VLF=1  angleLF=0
      settings: AttributesFormatString=|
      | %<ID>
      | %<Vbase>V
      | %<VLF>pu
      | %<angleLF>deg.
      | %<Name>
  bus7 : powerlib/Measurements/Load Flow Bus  LConnTagsString=a  ID=bus7  Vbase=110000  Vref=1  Vangle=0  VLF=1  angleLF=0
      settings: AttributesFormatString=|
      | %<ID>
      | %<Vbase>V
      | %<VLF>pu
      | %<angleLF>deg.
      | %<Name>
  bus70 : powerlib/Measurements/Load Flow Bus  LConnTagsString=a  ID=bus70  Vbase=220000  Vref=1  Vangle=0  VLF=1  angleLF=0
      settings: AttributesFormatString=|
      | %<ID>
      | %<Vbase>V
      | %<VLF>pu
      | %<angleLF>deg.
      | %<Name>
  bus71 : powerlib/Measurements/Load Flow Bus  LConnTagsString=a  ID=bus71  Vbase=220000  Vref=1  Vangle=0  VLF=1  angleLF=0
      settings: AttributesFormatString=|
      | %<ID>
      | %<Vbase>V
      | %<VLF>pu
      | %<angleLF>deg.
      | %<Name>
  bus72 : powerlib/Measurements/Load Flow Bus  LConnTagsString=a  ID=bus72  Vbase=220000  Vref=1  Vangle=0  VLF=1  angleLF=0
      settings: AttributesFormatString=|
      | %<ID>
      | %<Vbase>V
      | %<VLF>pu
      | %<angleLF>deg.
      | %<Name>
  bus73 : powerlib/Measurements/Load Flow Bus  LConnTagsString=a  ID=bus73  Vbase=220000  Vref=1  Vangle=0  VLF=1  angleLF=0
      settings: AttributesFormatString=|
      | %<ID>
      | %<Vbase>V
      | %<VLF>pu
      | %<angleLF>deg.
      | %<Name>
  bus74 : powerlib/Measurements/Load Flow Bus  LConnTagsString=a  ID=bus74  Vbase=220000  Vref=1  Vangle=0  VLF=1  angleLF=0
      settings: AttributesFormatString=|
      | %<ID>
      | %<Vbase>V
      | %<VLF>pu
      | %<angleLF>deg.
      | %<Name>
  bus75 : powerlib/Measurements/Load Flow Bus  LConnTagsString=a  ID=bus75  Vbase=220000  Vref=1  Vangle=0  VLF=1  angleLF=0
      settings: AttributesFormatString=|
      | %<ID>
      | %<Vbase>V
      | %<VLF>pu
      | %<angleLF>deg.
      | %<Name>
  bus76 : powerlib/Measurements/Load Flow Bus  LConnTagsString=a  ID=bus76  Vbase=220000  Vref=1  Vangle=0  VLF=1  angleLF=0
      settings: AttributesFormatString=|
      | %<ID>
      | %<Vbase>V
      | %<VLF>pu
      | %<angleLF>deg.
      | %<Name>
  bus77 : powerlib/Measurements/Load Flow Bus  LConnTagsString=a  ID=bus77  Vbase=220000  Vref=1  Vangle=0  VLF=1  angleLF=0
      settings: AttributesFormatString=|
      | %<ID>
      | %<Vbase>V
      | %<VLF>pu
      | %<angleLF>deg.
      | %<Name>
  bus78 : powerlib/Measurements/Load Flow Bus  LConnTagsString=a  ID=bus78  Vbase=220000  Vref=1  Vangle=0  VLF=1  angleLF=0
      settings: AttributesFormatString=|
      | %<ID>
      | %<Vbase>V
      | %<VLF>pu
      | %<angleLF>deg.
      | %<Name>
  bus79 : powerlib/Measurements/Load Flow Bus  LConnTagsString=a  ID=bus79  Vbase=220000  Vref=1  Vangle=0  VLF=1  angleLF=0
      settings: AttributesFormatString=|
      | %<ID>
      | %<Vbase>V
      | %<VLF>pu
      | %<angleLF>deg.
      | %<Name>
  bus8 : powerlib/Measurements/Load Flow Bus  LConnTagsString=a  ID=bus8  Vbase=110000  Vref=1  Vangle=0  VLF=1  angleLF=0
      settings: AttributesFormatString=|
      | %<ID>
      | %<Vbase>V
      | %<VLF>pu
      | %<angleLF>deg.
      | %<Name>
  bus80 : powerlib/Measurements/Load Flow Bus  LConnTagsString=a  ID=bus80  Vbase=220000  Vref=1  Vangle=0  VLF=1  angleLF=0
      settings: AttributesFormatString=|
      | %<ID>
      | %<Vbase>V
      | %<VLF>pu
      | %<angleLF>deg.
      | %<Name>
  bus81 : powerlib/Measurements/Load Flow Bus  LConnTagsString=a  ID=bus81  Vbase=220000  Vref=1  Vangle=0  VLF=1  angleLF=0
      settings: AttributesFormatString=|
      | %<ID>
      | %<Vbase>V
      | %<VLF>pu
      | %<angleLF>deg.
      | %<Name>
  bus82 : powerlib/Measurements/Load Flow Bus  LConnTagsString=a  ID=bus82  Vbase=220000  Vref=1  Vangle=0  VLF=1  angleLF=0
      settings: AttributesFormatString=|
      | %<ID>
      | %<Vbase>V
      | %<VLF>pu
      | %<angleLF>deg.
      | %<Name>
  bus83 : powerlib/Measurements/Load Flow Bus  LConnTagsString=a  ID=bus83  Vbase=220000  Vref=1  Vangle=0  VLF=1  angleLF=0
      settings: AttributesFormatString=|
      | %<ID>
      | %<Vbase>V
      | %<VLF>pu
      | %<angleLF>deg.
      | %<Name>
  bus84 : powerlib/Measurements/Load Flow Bus  LConnTagsString=a  ID=bus84  Vbase=220000  Vref=1  Vangle=0  VLF=1  angleLF=0
      settings: AttributesFormatString=|
      | %<ID>
      | %<Vbase>V
      | %<VLF>pu
      | %<angleLF>deg.
      | %<Name>
  bus85 : powerlib/Measurements/Load Flow Bus  LConnTagsString=a  ID=bus85  Vbase=220000  Vref=1  Vangle=0  VLF=1  angleLF=0
      settings: AttributesFormatString=|
      | %<ID>
      | %<Vbase>V
      | %<VLF>pu
      | %<angleLF>deg.
      | %<Name>
  bus86 : powerlib/Measurements/Load Flow Bus  LConnTagsString=a  ID=bus86  Vbase=220000  Vref=1  Vangle=0  VLF=1  angleLF=0
      settings: AttributesFormatString=|
      | %<ID>
      | %<Vbase>V
      | %<VLF>pu
      | %<angleLF>deg.
      | %<Name>
  bus87 : powerlib/Measurements/Load Flow Bus  LConnTagsString=a  ID=bus87  Vbase=220000  Vref=1  Vangle=0  VLF=1  angleLF=0
      settings: AttributesFormatString=|
      | %<ID>
      | %<Vbase>V
      | %<VLF>pu
      | %<angleLF>deg.
      | %<Name>
  bus88 : powerlib/Measurements/Load Flow Bus  LConnTagsString=a  ID=bus88  Vbase=220000  Vref=1  Vangle=0  VLF=1  angleLF=0
      settings: AttributesFormatString=|
      | %<ID>
      | %<Vbase>V
      | %<VLF>pu
      | %<angleLF>deg.
      | %<Name>
  bus89 : powerlib/Measurements/Load Flow Bus  LConnTagsString=a  ID=bus89  Vbase=220000  Vref=1  Vangle=0  VLF=1  angleLF=0
      settings: AttributesFormatString=|
      | %<ID>
      | %<Vbase>V
      | %<VLF>pu
      | %<angleLF>deg.
      | %<Name>
  bus9 : powerlib/Measurements/Load Flow Bus  LConnTagsString=a  ID=bus9  Vbase=110000  Vref=1  Vangle=0  VLF=1  angleLF=0
      settings: AttributesFormatString=|
      | %<ID>
      | %<Vbase>V
      | %<VLF>pu
      | %<angleLF>deg.
      | %<Name>
  bus90 : powerlib/Measurements/Load Flow Bus  LConnTagsString=a  ID=bus90  Vbase=220000  Vref=1  Vangle=0  VLF=1  angleLF=0
      settings: AttributesFormatString=|
      | %<ID>
      | %<Vbase>V
      | %<VLF>pu
      | %<angleLF>deg.
      | %<Name>
  bus91 : powerlib/Measurements/Load Flow Bus  LConnTagsString=a  ID=bus91  Vbase=220000  Vref=1  Vangle=0  VLF=1  angleLF=0
      settings: AttributesFormatString=|
      | %<ID>
      | %<Vbase>V
      | %<VLF>pu
      | %<angleLF>deg.
      | %<Name>
  bus92 : powerlib/Measurements/Load Flow Bus  LConnTagsString=a  ID=bus92  Vbase=220000  Vref=1  Vangle=0  VLF=1  angleLF=0
      settings: AttributesFormatString=|
      | %<ID>
      | %<Vbase>V
      | %<VLF>pu
      | %<angleLF>deg.
      | %<Name>
  bus93 : powerlib/Measurements/Load Flow Bus  LConnTagsString=a  ID=bus93  Vbase=220000  Vref=1  Vangle=0  VLF=1  angleLF=0
      settings: AttributesFormatString=|
      | %<ID>
      | %<Vbase>V
      | %<VLF>pu
      | %<angleLF>deg.
      | %<Name>
  bus94 : powerlib/Measurements/Load Flow Bus  LConnTagsString=a  ID=bus94  Vbase=220000  Vref=1  Vangle=0  VLF=1  angleLF=0
      settings: AttributesFormatString=|
      | %<ID>
      | %<Vbase>V
      | %<VLF>pu
      | %<angleLF>deg.
      | %<Name>
  bus95 : powerlib/Measurements/Load Flow Bus  LConnTagsString=a  ID=bus95  Vbase=220000  Vref=1  Vangle=0  VLF=1  angleLF=0
      settings: AttributesFormatString=|
      | %<ID>
      | %<Vbase>V
      | %<VLF>pu
      | %<angleLF>deg.
      | %<Name>
  bus96 : powerlib/Measurements/Load Flow Bus  LConnTagsString=a  ID=bus96  Vbase=220000  Vref=1  Vangle=0  VLF=1  angleLF=0
      settings: AttributesFormatString=|
      | %<ID>
      | %<Vbase>V
      | %<VLF>pu
      | %<angleLF>deg.
      | %<Name>
  bus97 : powerlib/Measurements/Load Flow Bus  LConnTagsString=a  ID=bus97  Vbase=220000  Vref=1  Vangle=0  VLF=1  angleLF=0
      settings: AttributesFormatString=|
      | %<ID>
      | %<Vbase>V
      | %<VLF>pu
      | %<angleLF>deg.
      | %<Name>
  bus98 : powerlib/Measurements/Load Flow Bus  LConnTagsString=a  ID=bus98  Vbase=220000  Vref=1  Vangle=0  VLF=1  angleLF=0
      settings: AttributesFormatString=|
      | %<ID>
      | %<Vbase>V
      | %<VLF>pu
      | %<angleLF>deg.
      | %<Name>
  bus99 : powerlib/Measurements/Load Flow Bus  LConnTagsString=a  ID=bus99  Vbase=220000  Vref=1  Vangle=0  VLF=1  angleLF=0
      settings: AttributesFormatString=|
      | %<ID>
      | %<Vbase>V
      | %<VLF>pu
      | %<angleLF>deg.
      | %<Name>
  powergui : powerlib/powergui  Priority=1  SimulationMode=Continuous  SolverType=Tustin  SampleTime=50e-6  frequency=60  SPID=off  DisableSnubberDevices=off  DisableRonSwitches=off  DisableVfSwitches=off  SwTol=0  Interpol=off  DisplayEquations=off  Ts=0  methode=off  frequencyindice=60  Pbase=100e6  ErrMax=1e-4  Iterations=50  UnitsV=kV  UnitsW=MW  FunctionMessages=off  echomessages=off  HookPort=off  EnableUseOfTLC=off  x0status=blocks  RestoreLinks=warning  ResistiveCurrentMeasurement=off  Frange=[0:2:500]  Ylog=off  Xlog=on  ShowGrid=off  save=off  variable=ZData  structure=0  ZoomFFT=off  StartTime=0.0  cycles=1  DisplayStyle=1  fundamental=60  FreqAxis=off  MaxFrequency=1000  frequencyindicesteady=1  RmsSteady=1  display=off
  connections:
  T_121436161__/LConn1 -- _CN_121436161_110000_CN_121431080_110000/LConn1
  T_121436161__/LConn2 -- _CN_121436161_110000_CN_121431080_110000/LConn2
  _CN_121436161_110000_CN_121431080_110000/LConn3 -- T_121436161__/LConn3 -- bus1/LConn1
  _CN_121436161_110000_CN_121431080_110000/RConn1 -- T_121431080__Sulfuros/RConn1 -- L_121431080/LConn1
  _CN_121436161_110000_CN_121431080_110000/RConn2 -- T_121431080__Sulfuros/RConn2 -- L_121431080/LConn2
  _CN_121436161_110000_CN_121431080_110000/RConn3 -- T_121431080__Sulfuros/RConn3 -- L_121431080/LConn3 -- bus2/LConn1
  _CN_119776135_110000_CN_119889425_110000/LConn1 -- T_119776135__/LConn1 -- _CN_119776135_110000_CN_95344808_110000/LConn1
  _CN_119776135_110000_CN_119889425_110000/LConn2 -- T_119776135__/LConn2 -- _CN_119776135_110000_CN_95344808_110000/LConn2
  _CN_119776135_110000_CN_119889425_110000/LConn3 -- T_119776135__/LConn3 -- _CN_119776135_110000_CN_95344808_110000/LConn3 -- bus3/LConn1
  _CN_119776135_110000_CN_119889425_110000/RConn1 -- T_119889425__/LConn1 -- _CN_119889425_110000_CN_95344808_110000/LConn1
  _CN_119776135_110000_CN_119889425_110000/RConn2 -- T_119889425__/LConn2 -- _CN_119889425_110000_CN_95344808_110000/LConn2
  _CN_119776135_110000_CN_119889425_110000/RConn3 -- T_119889425__/LConn3 -- _CN_119889425_110000_CN_95344808_110000/LConn3 -- bus4/LConn1
  _CN_119776135_110000_CN_95344808_110000/RConn1 -- T_95344808_220000;110000_Diego_de_Almagro/RConn1 -- _CN_119889425_110000_CN_95344808_110000/RConn1 -- L_95344808/LConn1
  _CN_119776135_110000_CN_95344808_110000/RConn2 -- T_95344808_220000;110000_Diego_de_Almagro/RConn2 -- _CN_119889425_110000_CN_95344808_110000/RConn2 -- L_95344808/LConn2
  _CN_119776135_110000_CN_95344808_110000/RConn3 -- T_95344808_220000;110000_Diego_de_Almagro/RConn3 -- _CN_119889425_110000_CN_95344808_110000/RConn3 -- L_95344808/LConn3 -- bus5/LConn1
  _CN_103247113_110000_CN_30455625_110000/LConn1 -- T_103247113__Subestación_El_Salto/RConn1 -- _CN_103247113_110000_CN_140087862_110000/LConn1 -- L_103247113/LConn1
  _CN_103247113_110000_CN_30455625_110000/LConn2 -- T_103247113__Subestación_El_Salto/RConn2 -- _CN_103247113_110000_CN_140087862_110000/LConn2 -- L_103247113/LConn2
  _CN_103247113_110000_CN_30455625_110000/LConn3 -- T_103247113__Subestación_El_Salto/RConn3 -- _CN_103247113_110000_CN_140087862_110000/LConn3 -- L_103247113/LConn3 -- bus6/LConn1
  T_30455625__SE_Los_Almendros/LConn1 -- _CN_103247113_110000_CN_30455625_110000/RConn1
  T_30455625__SE_Los_Almendros/LConn2 -- _CN_103247113_110000_CN_30455625_110000/RConn2
  _CN_103247113_110000_CN_30455625_110000/RConn3 -- T_30455625__SE_Los_Almendros/LConn3 -- bus7/LConn1
  T_140087862__Subestacion_Eléctrica_San_Cristobal/LConn1 -- _CN_103247113_110000_CN_140087862_110000/RConn1
  T_140087862__Subestacion_Eléctrica_San_Cristobal/LConn2 -- _CN_103247113_110000_CN_140087862_110000/RConn2
  _CN_103247113_110000_CN_140087862_110000/RConn3 -- T_140087862__Subestacion_Eléctrica_San_Cristobal/LConn3 -- bus8/LConn1
  _CN_121445146_110000_CN_321507700_110000/LConn1 -- T_121445146__Escondida/RConn1 -- L_121445146/LConn1
  _CN_121445146_110000_CN_321507700_110000/LConn2 -- T_121445146__Escondida/RConn2 -- L_121445146/LConn2
  _CN_121445146_110000_CN_321507700_110000/LConn3 -- T_121445146__Escondida/RConn3 -- L_121445146/LConn3 -- bus9/LConn1
  T_321507700__/LConn1 -- _CN_121445146_110000_CN_321507700_110000/RConn1
  T_321507700__/LConn2 -- _CN_121445146_110000_CN_321507700_110000/RConn2
  _CN_121445146_110000_CN_321507700_110000/RConn3 -- T_321507700__/LConn3 -- bus10/LConn1
  T_28321693__Subestación_San_Bernardo/LConn1 -- _CN_28321693_110000_CN_28321441_110000/LConn1
  T_28321693__Subestación_San_Bernardo/LConn2 -- _CN_28321693_110000_CN_28321441_110000/LConn2
  _CN_28321693_110000_CN_28321441_110000/LConn3 -- T_28321693__Subestación_San_Bernardo/LConn3 -- bus11/LConn1
  _CN_28321693_110000_CN_28321441_110000/RConn1 -- T_28321441__/LConn1 -- _CN_28321441_110000_CN_205950704_110000/LConn1
  _CN_28321693_110000_CN_28321441_110000/RConn2 -- T_28321441__/LConn2 -- _CN_28321441_110000_CN_205950704_110000/LConn2
  _CN_28321693_110000_CN_28321441_110000/RConn3 -- T_28321441__/LConn3 -- _CN_28321441_110000_CN_205950704_110000/LConn3 -- bus12/LConn1
  _CN_184250655_110000_CN_220292365_110000/LConn1 -- T_184250655__Subestación_Eléctrica_Cerro_Navia/RConn1 -- _CN_184250655_110000_CN_26409096_110000/LConn1 -- _CN_184250655_110000_CN_123910738_110000/LConn1 -- L_184250655/LConn1 -- _CN_184250655_110000_CN_394868441_110000/LConn1 -- _CN_184250655_110000_CN_48571065_110000/LConn1 -- _CN_184250655_110000_CN_94811802_110000/LConn1 -- _CN_184250655_110000_CN_236802012_110000/LConn1
  _CN_184250655_110000_CN_220292365_110000/LConn2 -- T_184250655__Subestación_Eléctrica_Cerro_Navia/RConn2 -- _CN_184250655_110000_CN_26409096_110000/LConn2 -- _CN_184250655_110000_CN_123910738_110000/LConn2 -- L_184250655/LConn2 -- _CN_184250655_110000_CN_394868441_110000/LConn2 -- _CN_184250655_110000_CN_48571065_110000/LConn2 -- _CN_184250655_110000_CN_94811802_110000/LConn2 -- _CN_184250655_110000_CN_236802012_110000/LConn2
  _CN_184250655_110000_CN_220292365_110000/LConn3 -- T_184250655__Subestación_Eléctrica_Cerro_Navia/RConn3 -- _CN_184250655_110000_CN_26409096_110000/LConn3 -- _CN_184250655_110000_CN_123910738_110000/LConn3 -- L_184250655/LConn3 -- bus13/LConn1 -- _CN_184250655_110000_CN_394868441_110000/LConn3 -- _CN_184250655_110000_CN_48571065_110000/LConn3 -- _CN_184250655_110000_CN_94811802_110000/LConn3 -- _CN_184250655_110000_CN_236802012_110000/LConn3
  T_220292365__/LConn1 -- _CN_184250655_110000_CN_220292365_110000/RConn1
  T_220292365__/LConn2 -- _CN_184250655_110000_CN_220292365_110000/RConn2
  _CN_184250655_110000_CN_220292365_110000/RConn3 -- T_220292365__/LConn3 -- bus14/LConn1
  T_394868441__/LConn1 -- _CN_184250655_110000_CN_394868441_110000/RConn1
  T_394868441__/LConn2 -- _CN_184250655_110000_CN_394868441_110000/RConn2
  _CN_184250655_110000_CN_394868441_110000/RConn3 -- T_394868441__/LConn3 -- bus15/LConn1
  _CN_184250655_110000_CN_48571065_110000/RConn1 -- T_48571065__/RConn1 -- _CN_48571065_110000_CN_194041555_110000/LConn1 -- L_48571065/LConn1
  _CN_184250655_110000_CN_48571065_110000/RConn2 -- T_48571065__/RConn2 -- _CN_48571065_110000_CN_194041555_110000/LConn2 -- L_48571065/LConn2
  _CN_184250655_110000_CN_48571065_110000/RConn3 -- T_48571065__/RConn3 -- _CN_48571065_110000_CN_194041555_110000/LConn3 -- L_48571065/LConn3 -- bus16/LConn1
  T_94811802__/LConn1 -- _CN_184250655_110000_CN_94811802_110000/RConn1
  T_94811802__/LConn2 -- _CN_184250655_110000_CN_94811802_110000/RConn2
  _CN_184250655_110000_CN_94811802_110000/RConn3 -- T_94811802__/LConn3 -- bus17/LConn1
  T_236802012__/LConn1 -- _CN_184250655_110000_CN_236802012_110000/RConn1
  T_236802012__/LConn2 -- _CN_184250655_110000_CN_236802012_110000/RConn2
  _CN_184250655_110000_CN_236802012_110000/RConn3 -- T_236802012__/LConn3 -- bus18/LConn1
  G_26409096_Termoeléctrica_Renca/RConn1 -- _CN_184250655_110000_CN_26409096_110000/RConn1
  G_26409096_Termoeléctrica_Renca/RConn2 -- _CN_184250655_110000_CN_26409096_110000/RConn2
  _CN_184250655_110000_CN_26409096_110000/RConn3 -- G_26409096_Termoeléctrica_Renca/RConn3 -- bus19/LConn1
  T_123910738__/LConn1 -- _CN_184250655_110000_CN_123910738_110000/RConn1
  T_123910738__/LConn2 -- _CN_184250655_110000_CN_123910738_110000/RConn2
  _CN_184250655_110000_CN_123910738_110000/RConn3 -- T_123910738__/LConn3 -- bus20/LConn1
  T_205950704__/LConn1 -- _CN_28321441_110000_CN_205950704_110000/RConn1
  T_205950704__/LConn2 -- _CN_28321441_110000_CN_205950704_110000/RConn2
  _CN_28321441_110000_CN_205950704_110000/RConn3 -- T_205950704__/LConn3 -- bus21/LConn1
  _CN_48571065_110000_CN_194041555_110000/RConn1 -- T_194041555__/LConn1 -- _CN_194041555_110000_CN_120227699_110000/LConn1 -- _CN_194041555_110000_CN_94815220_110000/LConn1
  _CN_48571065_110000_CN_194041555_110000/RConn2 -- T_194041555__/LConn2 -- _CN_194041555_110000_CN_120227699_110000/LConn2 -- _CN_194041555_110000_CN_94815220_110000/LConn2
  _CN_48571065_110000_CN_194041555_110000/RConn3 -- T_194041555__/LConn3 -- _CN_194041555_110000_CN_120227699_110000/LConn3 -- _CN_194041555_110000_CN_94815220_110000/LConn3 -- bus22/LConn1
  G_120227699_Subestacion_Ochagavia/RConn1 -- _CN_194041555_110000_CN_120227699_110000/RConn1
  G_120227699_Subestacion_Ochagavia/RConn2 -- _CN_194041555_110000_CN_120227699_110000/RConn2
  _CN_194041555_110000_CN_120227699_110000/RConn3 -- G_120227699_Subestacion_Ochagavia/RConn3 -- bus23/LConn1
  T_94815220__/LConn1 -- _CN_194041555_110000_CN_94815220_110000/RConn1
  T_94815220__/LConn2 -- _CN_194041555_110000_CN_94815220_110000/RConn2
  _CN_194041555_110000_CN_94815220_110000/RConn3 -- T_94815220__/LConn3 -- bus24/LConn1
  T_183356930__/LConn1 -- _CN_183356930_220000_CN_182692487_220000/LConn1
  T_183356930__/LConn2 -- _CN_183356930_220000_CN_182692487_220000/LConn2
  _CN_183356930_220000_CN_182692487_220000/LConn3 -- T_183356930__/LConn3 -- bus25/LConn1
  T_182692487__/LConn1 -- _CN_183356930_220000_CN_182692487_220000/RConn1
  T_182692487__/LConn2 -- _CN_183356930_220000_CN_182692487_220000/RConn2
  _CN_183356930_220000_CN_182692487_220000/RConn3 -- T_182692487__/LConn3 -- bus26/LConn1
  T_169337349__S_E_Angamos___Eléctrica_Angamos/LConn1 -- _CN_169337349_220000_CN_168851504_220000/LConn1
  T_169337349__S_E_Angamos___Eléctrica_Angamos/LConn2 -- _CN_169337349_220000_CN_168851504_220000/LConn2
  _CN_169337349_220000_CN_168851504_220000/LConn3 -- T_169337349__S_E_Angamos___Eléctrica_Angamos/LConn3 -- bus27/LConn1
  T_168851504__/LConn1 -- _CN_169337349_220000_CN_168851504_220000/RConn1
  T_168851504__/LConn2 -- _CN_169337349_220000_CN_168851504_220000/RConn2
  _CN_169337349_220000_CN_168851504_220000/RConn3 -- T_168851504__/LConn3 -- bus28/LConn1
  T_157553674__Subestacion_Pozo_Almonte/LConn1 -- _CN_157553674_220000_CN_182735456_220000/LConn1
  T_157553674__Subestacion_Pozo_Almonte/LConn2 -- _CN_157553674_220000_CN_182735456_220000/LConn2
  _CN_157553674_220000_CN_182735456_220000/LConn3 -- T_157553674__Subestacion_Pozo_Almonte/LConn3 -- bus29/LConn1
  _CN_157553674_220000_CN_182735456_220000/RConn1 -- T_182735456__S_E_Lagunas/LConn1 -- _CN_182735456_220000_CN_182692483_220000/LConn1 -- _CN_182735456_220000_CN_111486352_220000/LConn1
  _CN_157553674_220000_CN_182735456_220000/RConn2 -- T_182735456__S_E_Lagunas/LConn2 -- _CN_182735456_220000_CN_182692483_220000/LConn2 -- _CN_182735456_220000_CN_111486352_220000/LConn2
  _CN_157553674_220000_CN_182735456_220000/RConn3 -- T_182735456__S_E_Lagunas/LConn3 -- _CN_182735456_220000_CN_182692483_220000/LConn3 -- bus30/LConn1 -- _CN_182735456_220000_CN_111486352_220000/LConn3
  T_394165771__/LConn1 -- _CN_394165771_220000_CN_349891827_220000/LConn1
  T_394165771__/LConn2 -- _CN_394165771_220000_CN_349891827_220000/LConn2
  _CN_394165771_220000_CN_349891827_220000/LConn3 -- T_394165771__/LConn3 -- bus31/LConn1
  _CN_394165771_220000_CN_349891827_220000/RConn1 -- T_349891827__S_E_Polpaico/LConn1 -- _CN_349891827_220000_CN_123909946_220000/LConn1 -- _CN_349891827_220000_CN_27215229_220000/LConn1 -- _CN_236594201_220000_CN_349891827_220000/LConn1 -- _CN_140162733_220000_CN_349891827_220000/LConn1 -- _CN_349891826_220000_CN_349891827_220000/LConn1
  _CN_394165771_220000_CN_349891827_220000/RConn2 -- T_349891827__S_E_Polpaico/LConn2 -- _CN_349891827_220000_CN_123909946_220000/LConn2 -- _CN_349891827_220000_CN_27215229_220000/LConn2 -- _CN_236594201_220000_CN_349891827_220000/LConn2 -- _CN_140162733_220000_CN_349891827_220000/LConn2 -- _CN_349891826_220000_CN_349891827_220000/LConn2
  _CN_394165771_220000_CN_349891827_220000/RConn3 -- T_349891827__S_E_Polpaico/LConn3 -- _CN_349891827_220000_CN_123909946_220000/LConn3 -- bus32/LConn1 -- _CN_349891827_220000_CN_27215229_220000/LConn3 -- _CN_236594201_220000_CN_349891827_220000/LConn3 -- _CN_140162733_220000_CN_349891827_220000/LConn3 -- _CN_349891826_220000_CN_349891827_220000/LConn3
  _CN_236594201_220000_CN_349891827_220000/RConn1 -- T_236594201__/LConn1 -- _CN_236594201_220000_CN_184250655_220000/LConn1
  _CN_236594201_220000_CN_349891827_220000/RConn2 -- T_236594201__/LConn2 -- _CN_236594201_220000_CN_184250655_220000/LConn2
  _CN_236594201_220000_CN_349891827_220000/RConn3 -- T_236594201__/LConn3 -- _CN_236594201_220000_CN_184250655_220000/LConn3 -- bus33/LConn1
  _CN_236594201_220000_CN_184250655_220000/RConn1 -- T_184250655__Subestación_Eléctrica_Cerro_Navia/LConn1 -- _CN_48571065_220000_CN_184250655_220000/LConn1
  _CN_236594201_220000_CN_184250655_220000/RConn2 -- T_184250655__Subestación_Eléctrica_Cerro_Navia/LConn2 -- _CN_48571065_220000_CN_184250655_220000/LConn2
  _CN_236594201_220000_CN_184250655_220000/RConn3 -- T_184250655__Subestación_Eléctrica_Cerro_Navia/LConn3 -- _CN_48571065_220000_CN_184250655_220000/LConn3 -- bus34/LConn1
  T_121431080__Sulfuros/LConn1 -- _CN_121431080_220000_CN_121431104_220000/LConn1
  T_121431080__Sulfuros/LConn2 -- _CN_121431080_220000_CN_121431104_220000/LConn2
  _CN_121431080_220000_CN_121431104_220000/LConn3 -- T_121431080__Sulfuros/LConn3 -- bus35/LConn1
  _CN_121431080_220000_CN_121431104_220000/RConn1 -- T_121431104__Domeyko/LConn1 -- _CN_121431094_220000_CN_121431104_220000/LConn1 -- _CN_121431104_220000_CN_121455793_220000/LConn1
  _CN_121431080_220000_CN_121431104_220000/RConn2 -- T_121431104__Domeyko/LConn2 -- _CN_121431094_220000_CN_121431104_220000/LConn2 -- _CN_121431104_220000_CN_121455793_220000/LConn2
  _CN_121431080_220000_CN_121431104_220000/RConn3 -- T_121431104__Domeyko/LConn3 -- _CN_121431094_220000_CN_121431104_220000/LConn3 -- _CN_121431104_220000_CN_121455793_220000/LConn3 -- bus36/LConn1
  Cardones_Maitencillo_C3_CN_182235178_220000_CN_119834529_220000/LConn1 -- T_182235178__/LConn1 -- _CN_182235178_220000_CN_182236045_220000/LConn1 -- _CN_182235178_220000_CN_343069454_220000/LConn1
  Cardones_Maitencillo_C3_CN_182235178_220000_CN_119834529_220000/LConn2 -- T_182235178__/LConn2 -- _CN_182235178_220000_CN_182236045_220000/LConn2 -- _CN_182235178_220000_CN_343069454_220000/LConn2
  Cardones_Maitencillo_C3_CN_182235178_220000_CN_119834529_220000/LConn3 -- T_182235178__/LConn3 -- _CN_182235178_220000_CN_182236045_220000/LConn3 -- _CN_182235178_220000_CN_343069454_220000/LConn3 -- bus37/LConn1
  Cardones_Maitencillo_C3_CN_182235178_220000_CN_119834529_220000/RConn1 -- T_119834529__Cardones/LConn1 -- _CN_119688342_220000_CN_119834529_220000/LConn1 -- _CN_393463140_220000_CN_119834529_220000/LConn1
  Cardones_Maitencillo_C3_CN_182235178_220000_CN_119834529_220000/RConn2 -- T_119834529__Cardones/LConn2 -- _CN_119688342_220000_CN_119834529_220000/LConn2 -- _CN_393463140_220000_CN_119834529_220000/LConn2
  Cardones_Maitencillo_C3_CN_182235178_220000_CN_119834529_220000/RConn3 -- T_119834529__Cardones/LConn3 -- _CN_119688342_220000_CN_119834529_220000/LConn3 -- _CN_393463140_220000_CN_119834529_220000/LConn3 -- bus38/LConn1
  T_182236045__/LConn1 -- _CN_182235178_220000_CN_182236045_220000/RConn1
  T_182236045__/LConn2 -- _CN_182235178_220000_CN_182236045_220000/RConn2
  _CN_182235178_220000_CN_182236045_220000/RConn3 -- T_182236045__/LConn3 -- bus39/LConn1
  _CN_182235178_220000_CN_343069454_220000/RConn1 -- G_343069454_Parque_eólico_Punta_Colorada/RConn1 -- _CN_375149685_220000_CN_343069454_220000/LConn1
  _CN_182235178_220000_CN_343069454_220000/RConn2 -- G_343069454_Parque_eólico_Punta_Colorada/RConn2 -- _CN_375149685_220000_CN_343069454_220000/LConn2
  _CN_182235178_220000_CN_343069454_220000/RConn3 -- G_343069454_Parque_eólico_Punta_Colorada/RConn3 -- _CN_375149685_220000_CN_343069454_220000/LConn3 -- bus40/LConn1
  T_118304300__/LConn1 -- _CN_118304300_220000_CN_167666088_220000/LConn1
  T_118304300__/LConn2 -- _CN_118304300_220000_CN_167666088_220000/LConn2
  _CN_118304300_220000_CN_167666088_220000/LConn3 -- T_118304300__/LConn3 -- bus41/LConn1
  _CN_118304300_220000_CN_167666088_220000/RConn1 -- T_167666088__Subestación_Charrúa_(Paño_220_kV)/LConn1 -- S_E_Charrúa___S_E_Coronel_1x220_kV_CN_187680146_220000_CN_167666088_220000/LConn1 -- _CN_167666088_220000_CN_167666093_220000/LConn1 -- _CN_187201126_220000_CN_167666088_220000/LConn1 -- _CN_168492929_220000_CN_167666088_220000/LConn1 -- S_E_Mulchén___S_E_Charrúa_2x220_kV_CN_354354025_220000_CN_167666088_220000/LConn1 -- S_E_Antuco___S_E_Charrúa_2x220_kV_CN_200067463_220000_CN_167666088_220000/LConn1 -- S_E_Charrúa___S_E_Temuco_1x220_kV_CN_395644253_220000_CN_167666088_220000/LConn1
  _CN_118304300_220000_CN_167666088_220000/RConn2 -- T_167666088__Subestación_Charrúa_(Paño_220_kV)/LConn2 -- S_E_Charrúa___S_E_Coronel_1x220_kV_CN_187680146_220000_CN_167666088_220000/LConn2 -- _CN_167666088_220000_CN_167666093_220000/LConn2 -- _CN_187201126_220000_CN_167666088_220000/LConn2 -- _CN_168492929_220000_CN_167666088_220000/LConn2 -- S_E_Mulchén___S_E_Charrúa_2x220_kV_CN_354354025_220000_CN_167666088_220000/LConn2 -- S_E_Antuco___S_E_Charrúa_2x220_kV_CN_200067463_220000_CN_167666088_220000/LConn2 -- S_E_Charrúa___S_E_Temuco_1x220_kV_CN_395644253_220000_CN_167666088_220000/LConn2
  _CN_118304300_220000_CN_167666088_220000/RConn3 -- T_167666088__Subestación_Charrúa_(Paño_220_kV)/LConn3 -- S_E_Charrúa___S_E_Coronel_1x220_kV_CN_187680146_220000_CN_167666088_220000/LConn3 -- _CN_167666088_220000_CN_167666093_220000/LConn3 -- bus42/LConn1 -- _CN_187201126_220000_CN_167666088_220000/LConn3 -- _CN_168492929_220000_CN_167666088_220000/LConn3 -- S_E_Mulchén___S_E_Charrúa_2x220_kV_CN_354354025_220000_CN_167666088_220000/LConn3 -- S_E_Antuco___S_E_Charrúa_2x220_kV_CN_200067463_220000_CN_167666088_220000/LConn3 -- S_E_Charrúa___S_E_Temuco_1x220_kV_CN_395644253_220000_CN_167666088_220000/LConn3
  _CN_395644253_220000_CN_140002904_220000/LConn1 -- T_395644253__/LConn1 -- S_E_Charrúa___S_E_Temuco_1x220_kV_CN_395644253_220000_CN_120102647_220000/LConn1 -- S_E_Charrúa___S_E_Temuco_1x220_kV_CN_395644253_220000_CN_167666088_220000/RConn1
  _CN_395644253_220000_CN_140002904_220000/LConn2 -- T_395644253__/LConn2 -- S_E_Charrúa___S_E_Temuco_1x220_kV_CN_395644253_220000_CN_120102647_220000/LConn2 -- S_E_Charrúa___S_E_Temuco_1x220_kV_CN_395644253_220000_CN_167666088_220000/RConn2
  _CN_395644253_220000_CN_140002904_220000/LConn3 -- T_395644253__/LConn3 -- S_E_Charrúa___S_E_Temuco_1x220_kV_CN_395644253_220000_CN_120102647_220000/LConn3 -- S_E_Charrúa___S_E_Temuco_1x220_kV_CN_395644253_220000_CN_167666088_220000/RConn3 -- bus43/LConn1
  _CN_395644253_220000_CN_140002904_220000/RConn1 -- T_140002904__Temuco/LConn1 -- _CN_187100722_220000_CN_140002904_220000/LConn1
  _CN_395644253_220000_CN_140002904_220000/RConn2 -- T_140002904__Temuco/LConn2 -- _CN_187100722_220000_CN_140002904_220000/LConn2
  _CN_395644253_220000_CN_140002904_220000/RConn3 -- T_140002904__Temuco/LConn3 -- _CN_187100722_220000_CN_140002904_220000/LConn3 -- bus44/LConn1
  T_120102647__/LConn1 -- S_E_Charrúa___S_E_Temuco_1x220_kV_CN_395644253_220000_CN_120102647_220000/RConn1
  T_120102647__/LConn2 -- S_E_Charrúa___S_E_Temuco_1x220_kV_CN_395644253_220000_CN_120102647_220000/RConn2
  S_E_Charrúa___S_E_Temuco_1x220_kV_CN_395644253_220000_CN_120102647_220000/RConn3 -- T_120102647__/LConn3 -- bus45/LConn1
  _CN_187100722_220000_CN_140002904_220000/RConn1 -- T_187100722__S_E_Cautín/LConn1 -- _CN_187100722_220000_CN_190325675_220000/LConn1 -- _CN_187100722_220000_CN_182803372_220000/LConn1 -- S_E_Cautín___S_E_Mulchén_2x220_kV_CN_187100722_220000_CN_354354025_220000/LConn1
  _CN_187100722_220000_CN_140002904_220000/RConn2 -- T_187100722__S_E_Cautín/LConn2 -- _CN_187100722_220000_CN_190325675_220000/LConn2 -- _CN_187100722_220000_CN_182803372_220000/LConn2 -- S_E_Cautín___S_E_Mulchén_2x220_kV_CN_187100722_220000_CN_354354025_220000/LConn2
  _CN_187100722_220000_CN_140002904_220000/RConn3 -- T_187100722__S_E_Cautín/LConn3 -- _CN_187100722_220000_CN_190325675_220000/LConn3 -- _CN_187100722_220000_CN_182803372_220000/LConn3 -- S_E_Cautín___S_E_Mulchén_2x220_kV_CN_187100722_220000_CN_354354025_220000/LConn3 -- bus46/LConn1
  _CN_187100722_220000_CN_190325675_220000/RConn1 -- T_190325675__/LConn1 -- _CN_180536025_220000_CN_190325675_220000/LConn1
  _CN_187100722_220000_CN_190325675_220000/RConn2 -- T_190325675__/LConn2 -- _CN_180536025_220000_CN_190325675_220000/LConn2
  _CN_187100722_220000_CN_190325675_220000/RConn3 -- T_190325675__/LConn3 -- _CN_180536025_220000_CN_190325675_220000/LConn3 -- bus47/LConn1
  T_182803372__Valdivia/LConn1 -- _CN_187100722_220000_CN_182803372_220000/RConn1
  T_182803372__Valdivia/LConn2 -- _CN_187100722_220000_CN_182803372_220000/RConn2
  _CN_187100722_220000_CN_182803372_220000/RConn3 -- T_182803372__Valdivia/LConn3 -- bus48/LConn1
  S_E_Cautín___S_E_Mulchén_2x220_kV_CN_187100722_220000_CN_354354025_220000/RConn1 -- T_354354025__S_E_Mulchén/LConn1 -- S_E_Mulchén___S_E_Charrúa_2x220_kV_CN_354354025_220000_CN_167666088_220000/RConn1
  S_E_Cautín___S_E_Mulchén_2x220_kV_CN_187100722_220000_CN_354354025_220000/RConn2 -- T_354354025__S_E_Mulchén/LConn2 -- S_E_Mulchén___S_E_Charrúa_2x220_kV_CN_354354025_220000_CN_167666088_220000/RConn2
  S_E_Cautín___S_E_Mulchén_2x220_kV_CN_187100722_220000_CN_354354025_220000/RConn3 -- T_354354025__S_E_Mulchén/LConn3 -- S_E_Mulchén___S_E_Charrúa_2x220_kV_CN_354354025_220000_CN_167666088_220000/RConn3 -- bus49/LConn1
  _CN_121431094_220000_CN_30641904_220000/LConn1 -- T_121431094__/LConn1 -- _CN_121431094_220000_CN_121431104_220000/RConn1 -- _CN_121431094_220000_CN_121236949_220000/LConn1
  _CN_121431094_220000_CN_30641904_220000/LConn2 -- T_121431094__/LConn2 -- _CN_121431094_220000_CN_121431104_220000/RConn2 -- _CN_121431094_220000_CN_121236949_220000/LConn2
  _CN_121431094_220000_CN_30641904_220000/LConn3 -- T_121431094__/LConn3 -- _CN_121431094_220000_CN_121431104_220000/RConn3 -- bus50/LConn1 -- _CN_121431094_220000_CN_121236949_220000/LConn3
  _CN_121431094_220000_CN_30641904_220000/RConn1 -- T_30641904_110000_S_E_O'higgins/LConn1 -- _CN_30641904_220000_CN_120471866_220000/LConn1 -- _CN_120960385_220000_CN_30641904_220000/LConn1
  _CN_121431094_220000_CN_30641904_220000/RConn2 -- T_30641904_110000_S_E_O'higgins/LConn2 -- _CN_30641904_220000_CN_120471866_220000/LConn2 -- _CN_120960385_220000_CN_30641904_220000/LConn2
  _CN_121431094_220000_CN_30641904_220000/RConn3 -- T_30641904_110000_S_E_O'higgins/LConn3 -- _CN_30641904_220000_CN_120471866_220000/LConn3 -- bus51/LConn1 -- _CN_120960385_220000_CN_30641904_220000/LConn3
  T_121236949__/LConn1 -- _CN_121431094_220000_CN_121236949_220000/RConn1
  T_121236949__/LConn2 -- _CN_121431094_220000_CN_121236949_220000/RConn2
  _CN_121431094_220000_CN_121236949_220000/RConn3 -- T_121236949__/LConn3 -- bus52/LConn1
  T_200239163__/LConn1 -- _CN_200239163_220000_CN_200067463_220000/LConn1
  T_200239163__/LConn2 -- _CN_200239163_220000_CN_200067463_220000/LConn2
  _CN_200239163_220000_CN_200067463_220000/LConn3 -- T_200239163__/LConn3 -- bus53/LConn1
  _CN_200239163_220000_CN_200067463_220000/RConn1 -- T_200067463__/LConn1 -- S_E_Antuco___S_E_Charrúa_2x220_kV_CN_200067463_220000_CN_167666088_220000/RConn1
  _CN_200239163_220000_CN_200067463_220000/RConn2 -- T_200067463__/LConn2 -- S_E_Antuco___S_E_Charrúa_2x220_kV_CN_200067463_220000_CN_167666088_220000/RConn2
  _CN_200239163_220000_CN_200067463_220000/RConn3 -- T_200067463__/LConn3 -- S_E_Antuco___S_E_Charrúa_2x220_kV_CN_200067463_220000_CN_167666088_220000/RConn3 -- bus54/LConn1
  T_121455793__Lagunas_Seca/LConn1 -- _CN_121431104_220000_CN_121455793_220000/RConn1
  T_121455793__Lagunas_Seca/LConn2 -- _CN_121431104_220000_CN_121455793_220000/RConn2
  _CN_121431104_220000_CN_121455793_220000/RConn3 -- T_121455793__Lagunas_Seca/LConn3 -- bus55/LConn1
  _CN_328656452_220000_CN_30641628_220000/LConn1 -- T_328656452__S_E_Mantos_Blancos/LConn1 -- _CN_328656452_220000_CN_121623737_220000/LConn1 -- _CN_328656452_220000_CN_120712016_220000/LConn1
  _CN_328656452_220000_CN_30641628_220000/LConn2 -- T_328656452__S_E_Mantos_Blancos/LConn2 -- _CN_328656452_220000_CN_121623737_220000/LConn2 -- _CN_328656452_220000_CN_120712016_220000/LConn2
  _CN_328656452_220000_CN_30641628_220000/LConn3 -- T_328656452__S_E_Mantos_Blancos/LConn3 -- _CN_328656452_220000_CN_121623737_220000/LConn3 -- bus56/LConn1 -- _CN_328656452_220000_CN_120712016_220000/LConn3
  _CN_328656452_220000_CN_30641628_220000/RConn1 -- T_30641628__S_E_Chacaya/LConn1 -- Línea_220_kV_Chacaya___El_Cobre_144_km_350_MVA_CN_168852850_220000_CN_30641628_220000/LConn1 -- _CN_120960385_220000_CN_30641628_220000/LConn1
  _CN_328656452_220000_CN_30641628_220000/RConn2 -- T_30641628__S_E_Chacaya/LConn2 -- Línea_220_kV_Chacaya___El_Cobre_144_km_350_MVA_CN_168852850_220000_CN_30641628_220000/LConn2 -- _CN_120960385_220000_CN_30641628_220000/LConn2
  _CN_328656452_220000_CN_30641628_220000/RConn3 -- T_30641628__S_E_Chacaya/LConn3 -- Línea_220_kV_Chacaya___El_Cobre_144_km_350_MVA_CN_168852850_220000_CN_30641628_220000/LConn3 -- bus57/LConn1 -- _CN_120960385_220000_CN_30641628_220000/LConn3
  T_120712016__S_E_Capricornio/LConn1 -- _CN_328656452_220000_CN_120712016_220000/RConn1
  T_120712016__S_E_Capricornio/LConn2 -- _CN_328656452_220000_CN_120712016_220000/RConn2
  _CN_328656452_220000_CN_120712016_220000/RConn3 -- T_120712016__S_E_Capricornio/LConn3 -- bus58/LConn1
  _CN_328656452_220000_CN_121623737_220000/RConn1 -- T_121623737__Laberinto/LConn1 -- _CN_121623737_220000_CN_168852850_220000/LConn1 -- _CN_121623737_220000_CN_136149844_220000/LConn1 -- _CN_121623737_220000_CN_170073895_220000/LConn1 -- _CN_121623737_220000_CN_121454923_220000/LConn1 -- _CN_121623737_220000_CN_121445157_220000/LConn1 -- _CN_121623737_220000_CN_321511794_220000/LConn1 -- _CN_121623737_220000_CN_121445146_220000/LConn1 -- _CN_121623737_220000_CN_111486352_220000/LConn1 -- _CN_121623737_220000_CN_321520065_220000/LConn1
  _CN_328656452_220000_CN_121623737_220000/RConn2 -- T_121623737__Laberinto/LConn2 -- _CN_121623737_220000_CN_168852850_220000/LConn2 -- _CN_121623737_220000_CN_136149844_220000/LConn2 -- _CN_121623737_220000_CN_170073895_220000/LConn2 -- _CN_121623737_220000_CN_121454923_220000/LConn2 -- _CN_121623737_220000_CN_121445157_220000/LConn2 -- _CN_121623737_220000_CN_321511794_220000/LConn2 -- _CN_121623737_220000_CN_121445146_220000/LConn2 -- _CN_121623737_220000_CN_111486352_220000/LConn2 -- _CN_121623737_220000_CN_321520065_220000/LConn2
  _CN_328656452_220000_CN_121623737_220000/RConn3 -- T_121623737__Laberinto/LConn3 -- _CN_121623737_220000_CN_168852850_220000/LConn3 -- _CN_121623737_220000_CN_136149844_220000/LConn3 -- _CN_121623737_220000_CN_170073895_220000/LConn3 -- bus59/LConn1 -- _CN_121623737_220000_CN_121454923_220000/LConn3 -- _CN_121623737_220000_CN_121445157_220000/LConn3 -- _CN_121623737_220000_CN_321511794_220000/LConn3 -- _CN_121623737_220000_CN_121445146_220000/LConn3 -- _CN_121623737_220000_CN_111486352_220000/LConn3 -- _CN_121623737_220000_CN_321520065_220000/LConn3
  T_145413703__/LConn1 -- _CN_145413703_220000_CN_24411638_220000/LConn1
  T_145413703__/LConn2 -- _CN_145413703_220000_CN_24411638_220000/LConn2
  _CN_145413703_220000_CN_24411638_220000/LConn3 -- T_145413703__/LConn3 -- bus60/LConn1
  T_24411638__Sub_Estacion_Melipulli/LConn1 -- _CN_145413703_220000_CN_24411638_220000/RConn1
  T_24411638__Sub_Estacion_Melipulli/LConn2 -- _CN_145413703_220000_CN_24411638_220000/RConn2
  _CN_145413703_220000_CN_24411638_220000/RConn3 -- T_24411638__Sub_Estacion_Melipulli/LConn3 -- bus61/LConn1
  _CN_170017864_220000_CN_111486352_220000/LConn1 -- T_170017864__S_E_El_Abra/LConn1 -- _CN_170017864_220000_CN_328652522_220000/LConn1
  _CN_170017864_220000_CN_111486352_220000/LConn2 -- T_170017864__S_E_El_Abra/LConn2 -- _CN_170017864_220000_CN_328652522_220000/LConn2
  _CN_170017864_220000_CN_111486352_220000/LConn3 -- T_170017864__S_E_El_Abra/LConn3 -- _CN_170017864_220000_CN_328652522_220000/LConn3 -- bus62/LConn1
  _CN_170017864_220000_CN_111486352_220000/RConn1 -- T_111486352__S_E_Crucero/LConn1 -- _CN_121623737_220000_CN_111486352_220000/RConn1 -- _CN_182735456_220000_CN_111486352_220000/RConn1 -- _CN_111486348_220000_CN_111486352_220000/LConn1
  _CN_170017864_220000_CN_111486352_220000/RConn2 -- T_111486352__S_E_Crucero/LConn2 -- _CN_121623737_220000_CN_111486352_220000/RConn2 -- _CN_182735456_220000_CN_111486352_220000/RConn2 -- _CN_111486348_220000_CN_111486352_220000/LConn2
  _CN_170017864_220000_CN_111486352_220000/RConn3 -- T_111486352__S_E_Crucero/LConn3 -- _CN_121623737_220000_CN_111486352_220000/RConn3 -- _CN_182735456_220000_CN_111486352_220000/RConn3 -- _CN_111486348_220000_CN_111486352_220000/LConn3 -- bus63/LConn1
  T_328652522__S_E_Rodomiro_Tomic/LConn1 -- _CN_170017864_220000_CN_328652522_220000/RConn1
  T_328652522__S_E_Rodomiro_Tomic/LConn2 -- _CN_170017864_220000_CN_328652522_220000/RConn2
  _CN_170017864_220000_CN_328652522_220000/RConn3 -- T_328652522__S_E_Rodomiro_Tomic/LConn3 -- bus64/LConn1
  T_48571065__/LConn1 -- _CN_48571065_220000_CN_184250655_220000/RConn1
  T_48571065__/LConn2 -- _CN_48571065_220000_CN_184250655_220000/RConn2
  _CN_48571065_220000_CN_184250655_220000/RConn3 -- T_48571065__/LConn3 -- bus65/LConn1
  T_121454923__Nueva_Zaldivar/LConn1 -- _CN_121623737_220000_CN_121454923_220000/RConn1
  T_121454923__Nueva_Zaldivar/LConn2 -- _CN_121623737_220000_CN_121454923_220000/RConn2
  _CN_121623737_220000_CN_121454923_220000/RConn3 -- T_121454923__Nueva_Zaldivar/LConn3 -- bus66/LConn1
  T_121445157__P__Óxidos/LConn1 -- _CN_121623737_220000_CN_121445157_220000/RConn1
  T_121445157__P__Óxidos/LConn2 -- _CN_121623737_220000_CN_121445157_220000/RConn2
  _CN_121623737_220000_CN_121445157_220000/RConn3 -- T_121445157__P__Óxidos/LConn3 -- bus67/LConn1
  T_321511794__Zaldivar/LConn1 -- _CN_121623737_220000_CN_321511794_220000/RConn1
  T_321511794__Zaldivar/LConn2 -- _CN_121623737_220000_CN_321511794_220000/RConn2
  _CN_121623737_220000_CN_321511794_220000/RConn3 -- T_321511794__Zaldivar/LConn3 -- bus68/LConn1
  T_121445146__Escondida/LConn1 -- _CN_121623737_220000_CN_121445146_220000/RConn1
  T_121445146__Escondida/LConn2 -- _CN_121623737_220000_CN_121445146_220000/RConn2
  _CN_121623737_220000_CN_121445146_220000/RConn3 -- T_121445146__Escondida/LConn3 -- bus69/LConn1
  T_321520065__Lomas_Bayas/LConn1 -- _CN_121623737_220000_CN_321520065_220000/RConn1
  T_321520065__Lomas_Bayas/LConn2 -- _CN_121623737_220000_CN_321520065_220000/RConn2
  _CN_121623737_220000_CN_321520065_220000/RConn3 -- T_321520065__Lomas_Bayas/LConn3 -- bus70/LConn1
  _CN_121623737_220000_CN_168852850_220000/RConn1 -- T_168852850__S_E_El_Cobre/LConn1 -- Línea_220_kV_El_Cobre_Gaby_57_km_189_MVA_CN_168852850_220000_CN_170066365_220000/LConn1 -- _CN_170022526_220000_CN_168852850_220000/LConn1 -- Línea_220_kV_Chacaya___El_Cobre_144_km_350_MVA_CN_168852850_220000_CN_30641628_220000/RConn1
  _CN_121623737_220000_CN_168852850_220000/RConn2 -- T_168852850__S_E_El_Cobre/LConn2 -- Línea_220_kV_El_Cobre_Gaby_57_km_189_MVA_CN_168852850_220000_CN_170066365_220000/LConn2 -- _CN_170022526_220000_CN_168852850_220000/LConn2 -- Línea_220_kV_Chacaya___El_Cobre_144_km_350_MVA_CN_168852850_220000_CN_30641628_220000/RConn2
  _CN_121623737_220000_CN_168852850_220000/RConn3 -- T_168852850__S_E_El_Cobre/LConn3 -- Línea_220_kV_El_Cobre_Gaby_57_km_189_MVA_CN_168852850_220000_CN_170066365_220000/LConn3 -- bus71/LConn1 -- _CN_170022526_220000_CN_168852850_220000/LConn3 -- Línea_220_kV_Chacaya___El_Cobre_144_km_350_MVA_CN_168852850_220000_CN_30641628_220000/RConn3
  T_136149844__Abengoa/LConn1 -- _CN_121623737_220000_CN_136149844_220000/RConn1
  T_136149844__Abengoa/LConn2 -- _CN_121623737_220000_CN_136149844_220000/RConn2
  _CN_121623737_220000_CN_136149844_220000/RConn3 -- T_136149844__Abengoa/LConn3 -- bus72/LConn1
  T_170073895__Oeste/LConn1 -- _CN_121623737_220000_CN_170073895_220000/RConn1
  T_170073895__Oeste/LConn2 -- _CN_121623737_220000_CN_170073895_220000/RConn2
  _CN_121623737_220000_CN_170073895_220000/RConn3 -- T_170073895__Oeste/LConn3 -- bus73/LConn1
  _CN_182735456_220000_CN_182692483_220000/RConn1 -- T_182692483__/LConn1 -- _CN_182692483_220000_CN_182747576_220000/LConn1 -- _CN_182692483_220000_CN_111486348_220000/LConn1
  _CN_182735456_220000_CN_182692483_220000/RConn2 -- T_182692483__/LConn2 -- _CN_182692483_220000_CN_182747576_220000/LConn2 -- _CN_182692483_220000_CN_111486348_220000/LConn2
  _CN_182735456_220000_CN_182692483_220000/RConn3 -- T_182692483__/LConn3 -- _CN_182692483_220000_CN_182747576_220000/LConn3 -- _CN_182692483_220000_CN_111486348_220000/LConn3 -- bus74/LConn1
  T_187201126__/LConn1 -- _CN_187201126_220000_CN_167666088_220000/RConn1
  T_187201126__/LConn2 -- _CN_187201126_220000_CN_167666088_220000/RConn2
  _CN_187201126_220000_CN_167666088_220000/RConn3 -- T_187201126__/LConn3 -- bus75/LConn1
  _CN_375149685_220000_CN_343046589_220000/LConn1 -- T_375149685__/LConn1 -- _CN_375149685_220000_CN_393489602_220000/LConn1 -- _CN_375149685_220000_CN_343069454_220000/RConn1
  _CN_375149685_220000_CN_343046589_220000/LConn2 -- T_375149685__/LConn2 -- _CN_375149685_220000_CN_393489602_220000/LConn2 -- _CN_375149685_220000_CN_343069454_220000/RConn2
  _CN_375149685_220000_CN_343046589_220000/LConn3 -- T_375149685__/LConn3 -- _CN_375149685_220000_CN_393489602_220000/LConn3 -- _CN_375149685_220000_CN_343069454_220000/RConn3 -- bus76/LConn1
  _CN_375149685_220000_CN_343046589_220000/RConn1 -- G_343046589_Parque_Eólico_Monte_Redondo/RConn1 -- _CN_393489604_220000_CN_343046589_220000/LConn1 -- _CN_219477643_220000_CN_343046589_220000/LConn1
  _CN_375149685_220000_CN_343046589_220000/RConn2 -- G_343046589_Parque_Eólico_Monte_Redondo/RConn2 -- _CN_393489604_220000_CN_343046589_220000/LConn2 -- _CN_219477643_220000_CN_343046589_220000/LConn2
  _CN_375149685_220000_CN_343046589_220000/RConn3 -- G_343046589_Parque_Eólico_Monte_Redondo/RConn3 -- _CN_393489604_220000_CN_343046589_220000/LConn3 -- bus77/LConn1 -- _CN_219477643_220000_CN_343046589_220000/LConn3
  T_393489602__/LConn1 -- _CN_375149685_220000_CN_393489602_220000/RConn1
  T_393489602__/LConn2 -- _CN_375149685_220000_CN_393489602_220000/RConn2
  _CN_375149685_220000_CN_393489602_220000/RConn3 -- T_393489602__/LConn3 -- bus78/LConn1
  _CN_170022524_220000_CN_170022526_220000/LConn1 -- T_170022524__El_Tesoro/LConn1 -- _CN_170022524_220000_CN_111486348_220000/LConn1
  _CN_170022524_220000_CN_170022526_220000/LConn2 -- T_170022524__El_Tesoro/LConn2 -- _CN_170022524_220000_CN_111486348_220000/LConn2
  _CN_170022524_220000_CN_170022526_220000/LConn3 -- T_170022524__El_Tesoro/LConn3 -- _CN_170022524_220000_CN_111486348_220000/LConn3 -- bus79/LConn1
  _CN_170022524_220000_CN_170022526_220000/RConn1 -- T_170022526__Esperanza/LConn1 -- _CN_170022526_220000_CN_168852850_220000/RConn1
  _CN_170022524_220000_CN_170022526_220000/RConn2 -- T_170022526__Esperanza/LConn2 -- _CN_170022526_220000_CN_168852850_220000/RConn2
  _CN_170022524_220000_CN_170022526_220000/RConn3 -- T_170022526__Esperanza/LConn3 -- _CN_170022526_220000_CN_168852850_220000/RConn3 -- bus80/LConn1
  _CN_170022524_220000_CN_111486348_220000/RConn1 -- T_111486348__S_E_Encuentro/LConn1 -- _CN_182692483_220000_CN_111486348_220000/RConn1 -- _CN_170023614_220000_CN_111486348_220000/LConn1 -- _CN_120860874_220000_CN_111486348_220000/LConn1 -- _CN_111486348_220000_CN_111486352_220000/RConn1
  _CN_170022524_220000_CN_111486348_220000/RConn2 -- T_111486348__S_E_Encuentro/LConn2 -- _CN_182692483_220000_CN_111486348_220000/RConn2 -- _CN_170023614_220000_CN_111486348_220000/LConn2 -- _CN_120860874_220000_CN_111486348_220000/LConn2 -- _CN_111486348_220000_CN_111486352_220000/RConn2
  _CN_170022524_220000_CN_111486348_220000/RConn3 -- T_111486348__S_E_Encuentro/LConn3 -- _CN_182692483_220000_CN_111486348_220000/RConn3 -- _CN_170023614_220000_CN_111486348_220000/LConn3 -- _CN_120860874_220000_CN_111486348_220000/LConn3 -- _CN_111486348_220000_CN_111486352_220000/RConn3 -- bus81/LConn1
  T_182747576__S_E_Quebrada_blanca/LConn1 -- _CN_182692483_220000_CN_182747576_220000/RConn1
  T_182747576__S_E_Quebrada_blanca/LConn2 -- _CN_182692483_220000_CN_182747576_220000/RConn2
  _CN_182692483_220000_CN_182747576_220000/RConn3 -- T_182747576__S_E_Quebrada_blanca/LConn3 -- bus82/LConn1
  T_226755205_220000_Paposo/LConn1 -- _CN_226755205_220000_CN_95344808_220000/LConn1
  T_226755205_220000_Paposo/LConn2 -- _CN_226755205_220000_CN_95344808_220000/LConn2
  _CN_226755205_220000_CN_95344808_220000/LConn3 -- T_226755205_220000_Paposo/LConn3 -- bus83/LConn1
  _CN_226755205_220000_CN_95344808_220000/RConn1 -- T_95344808_220000;110000_Diego_de_Almagro/LConn1 -- _CN_119688342_220000_CN_95344808_220000/LConn1
  _CN_226755205_220000_CN_95344808_220000/RConn2 -- T_95344808_220000;110000_Diego_de_Almagro/LConn2 -- _CN_119688342_220000_CN_95344808_220000/LConn2
  _CN_226755205_220000_CN_95344808_220000/RConn3 -- T_95344808_220000;110000_Diego_de_Almagro/LConn3 -- _CN_119688342_220000_CN_95344808_220000/LConn3 -- bus84/LConn1
  T_219477643__Central_Canela_II/LConn1 -- _CN_219477643_220000_CN_343046589_220000/RConn1
  T_219477643__Central_Canela_II/LConn2 -- _CN_219477643_220000_CN_343046589_220000/RConn2
  _CN_219477643_220000_CN_343046589_220000/RConn3 -- T_219477643__Central_Canela_II/LConn3 -- bus85/LConn1
  _CN_119688342_220000_CN_253852513_220000/LConn1 -- T_119688342__Carrera_Pinto/LConn1 -- _CN_119688342_220000_CN_119834529_220000/RConn1 -- _CN_119688342_220000_CN_95344808_220000/RConn1
  _CN_119688342_220000_CN_253852513_220000/LConn2 -- T_119688342__Carrera_Pinto/LConn2 -- _CN_119688342_220000_CN_119834529_220000/RConn2 -- _CN_119688342_220000_CN_95344808_220000/RConn2
  _CN_119688342_220000_CN_253852513_220000/LConn3 -- T_119688342__Carrera_Pinto/LConn3 -- _CN_119688342_220000_CN_119834529_220000/RConn3 -- _CN_119688342_220000_CN_95344808_220000/RConn3 -- bus86/LConn1
  T_253852513__/LConn1 -- _CN_119688342_220000_CN_253852513_220000/RConn1
  T_253852513__/LConn2 -- _CN_119688342_220000_CN_253852513_220000/RConn2
  _CN_119688342_220000_CN_253852513_220000/RConn3 -- T_253852513__/LConn3 -- bus87/LConn1
  T_140162733__/LConn1 -- _CN_140162733_220000_CN_349891827_220000/RConn1
  T_140162733__/LConn2 -- _CN_140162733_220000_CN_349891827_220000/RConn2
  _CN_140162733_220000_CN_349891827_220000/RConn3 -- T_140162733__/LConn3 -- bus88/LConn1
  T_170023614__/LConn1 -- _CN_170023614_220000_CN_111486348_220000/RConn1
  T_170023614__/LConn2 -- _CN_170023614_220000_CN_111486348_220000/RConn2
  _CN_170023614_220000_CN_111486348_220000/RConn3 -- T_170023614__/LConn3 -- bus89/LConn1
  T_393489604__/LConn1 -- _CN_393489604_220000_CN_343046589_220000/RConn1
  T_393489604__/LConn2 -- _CN_393489604_220000_CN_343046589_220000/RConn2
  _CN_393489604_220000_CN_343046589_220000/RConn3 -- T_393489604__/LConn3 -- bus90/LConn1
  _CN_120860874_220000_CN_120707837_220000/LConn1 -- T_120860874__S_E_Atacama/LConn1 -- _CN_120860874_220000_CN_111486348_220000/RConn1
  _CN_120860874_220000_CN_120707837_220000/LConn2 -- T_120860874__S_E_Atacama/LConn2 -- _CN_120860874_220000_CN_111486348_220000/RConn2
  _CN_120860874_220000_CN_120707837_220000/LConn3 -- T_120860874__S_E_Atacama/LConn3 -- _CN_120860874_220000_CN_111486348_220000/RConn3 -- bus91/LConn1
  T_120707837__/LConn1 -- _CN_120860874_220000_CN_120707837_220000/RConn1
  T_120707837__/LConn2 -- _CN_120860874_220000_CN_120707837_220000/RConn2
  _CN_120860874_220000_CN_120707837_220000/RConn3 -- T_120707837__/LConn3 -- bus92/LConn1
  _CN_120960385_220000_CN_30641628_220000/RConn1 -- T_120960385__S_E_Mejillones/LConn1 -- _CN_120960385_220000_CN_30641904_220000/RConn1
  _CN_120960385_220000_CN_30641628_220000/RConn2 -- T_120960385__S_E_Mejillones/LConn2 -- _CN_120960385_220000_CN_30641904_220000/RConn2
  _CN_120960385_220000_CN_30641628_220000/RConn3 -- T_120960385__S_E_Mejillones/LConn3 -- _CN_120960385_220000_CN_30641904_220000/RConn3 -- bus93/LConn1
  T_88147668__/LConn1 -- _CN_88147668_220000_CN_110804340_220000/LConn1
  T_88147668__/LConn2 -- _CN_88147668_220000_CN_110804340_220000/LConn2
  _CN_88147668_220000_CN_110804340_220000/LConn3 -- T_88147668__/LConn3 -- bus94/LConn1
  _CN_88147668_220000_CN_110804340_220000/RConn1 -- T_110804340__S_E_Condores/LConn1 -- _CN_110801625_220000_CN_110804340_220000/LConn1
  _CN_88147668_220000_CN_110804340_220000/RConn2 -- T_110804340__S_E_Condores/LConn2 -- _CN_110801625_220000_CN_110804340_220000/LConn2
  _CN_88147668_220000_CN_110804340_220000/RConn3 -- T_110804340__S_E_Condores/LConn3 -- _CN_110801625_220000_CN_110804340_220000/LConn3 -- bus95/LConn1
  T_180536025__/LConn1 -- _CN_180536025_220000_CN_190325675_220000/RConn1
  T_180536025__/LConn2 -- _CN_180536025_220000_CN_190325675_220000/RConn2
  _CN_180536025_220000_CN_190325675_220000/RConn3 -- T_180536025__/LConn3 -- bus96/LConn1
  T_120471866__Coloso_220_kV/LConn1 -- _CN_30641904_220000_CN_120471866_220000/RConn1
  T_120471866__Coloso_220_kV/LConn2 -- _CN_30641904_220000_CN_120471866_220000/RConn2
  _CN_30641904_220000_CN_120471866_220000/RConn3 -- T_120471866__Coloso_220_kV/LConn3 -- bus97/LConn1
  T_184191729__/LConn1 -- _CN_184191729_220000_CN_184197597_220000/LConn1
  T_184191729__/LConn2 -- _CN_184191729_220000_CN_184197597_220000/LConn2
  _CN_184191729_220000_CN_184197597_220000/LConn3 -- T_184191729__/LConn3 -- bus98/LConn1
  T_184197597__/LConn1 -- _CN_184191729_220000_CN_184197597_220000/RConn1
  T_184197597__/LConn2 -- _CN_184191729_220000_CN_184197597_220000/RConn2
  _CN_184191729_220000_CN_184197597_220000/RConn3 -- T_184197597__/LConn3 -- bus99/LConn1
  T_349891826__S_E_Polpaico/LConn1 -- _CN_349891826_220000_CN_349891827_220000/RConn1
  T_349891826__S_E_Polpaico/LConn2 -- _CN_349891826_220000_CN_349891827_220000/RConn2
  _CN_349891826_220000_CN_349891827_220000/RConn3 -- T_349891826__S_E_Polpaico/LConn3 -- bus100/LConn1
  _CN_349891827_220000_CN_27215229_220000/RConn1 -- T_27215229__/LConn1 -- _CN_27215229_220000_CN_27215745_220000/LConn1
  _CN_349891827_220000_CN_27215229_220000/RConn2 -- T_27215229__/LConn2 -- _CN_27215229_220000_CN_27215745_220000/LConn2
  _CN_349891827_220000_CN_27215229_220000/RConn3 -- T_27215229__/LConn3 -- _CN_27215229_220000_CN_27215745_220000/LConn3 -- bus101/LConn1
  _CN_349891827_220000_CN_123909946_220000/RConn1 -- T_123909946__/LConn1 -- _CN_103247113_220000_CN_123909946_220000/LConn1
  _CN_349891827_220000_CN_123909946_220000/RConn2 -- T_123909946__/LConn2 -- _CN_103247113_220000_CN_123909946_220000/LConn2
  _CN_349891827_220000_CN_123909946_220000/RConn3 -- T_123909946__/LConn3 -- _CN_103247113_220000_CN_123909946_220000/LConn3 -- bus102/LConn1
  T_155008260__/LConn1 -- _CN_155008260_220000_CN_91655961_220000/LConn1
  T_155008260__/LConn2 -- _CN_155008260_220000_CN_91655961_220000/LConn2
  _CN_155008260_220000_CN_91655961_220000/LConn3 -- T_155008260__/LConn3 -- bus103/LConn1
  T_91655961_220000_Subestacion_Electrica_Los_Vilos/LConn1 -- _CN_155008260_220000_CN_91655961_220000/RConn1
  T_91655961_220000_Subestacion_Electrica_Los_Vilos/LConn2 -- _CN_155008260_220000_CN_91655961_220000/RConn2
  _CN_155008260_220000_CN_91655961_220000/RConn3 -- T_91655961_220000_Subestacion_Electrica_Los_Vilos/LConn3 -- bus104/LConn1
  T_103247113__Subestación_El_Salto/LConn1 -- _CN_103247113_220000_CN_123909946_220000/RConn1
  T_103247113__Subestación_El_Salto/LConn2 -- _CN_103247113_220000_CN_123909946_220000/RConn2
  _CN_103247113_220000_CN_123909946_220000/RConn3 -- T_103247113__Subestación_El_Salto/LConn3 -- bus105/LConn1
  T_120791316__S_E_Esmeralda/LConn1 -- _CN_120791316_220000_CN_120791326_220000/LConn1
  T_120791316__S_E_Esmeralda/LConn2 -- _CN_120791316_220000_CN_120791326_220000/LConn2
  _CN_120791316_220000_CN_120791326_220000/LConn3 -- T_120791316__S_E_Esmeralda/LConn3 -- bus106/LConn1
  T_120791326__S_E_Esmeralda_Centro/LConn1 -- _CN_120791316_220000_CN_120791326_220000/RConn1
  T_120791326__S_E_Esmeralda_Centro/LConn2 -- _CN_120791316_220000_CN_120791326_220000/RConn2
  _CN_120791316_220000_CN_120791326_220000/RConn3 -- T_120791326__S_E_Esmeralda_Centro/LConn3 -- bus107/LConn1
  T_110801625__Tarapacá/LConn1 -- _CN_110801625_220000_CN_110804340_220000/RConn1
  T_110801625__Tarapacá/LConn2 -- _CN_110801625_220000_CN_110804340_220000/RConn2
  _CN_110801625_220000_CN_110804340_220000/RConn3 -- T_110801625__Tarapacá/LConn3 -- bus108/LConn1
  T_168492929__/LConn1 -- _CN_168492929_220000_CN_167666088_220000/RConn1
  T_168492929__/LConn2 -- _CN_168492929_220000_CN_167666088_220000/RConn2
  _CN_168492929_220000_CN_167666088_220000/RConn3 -- T_168492929__/LConn3 -- bus109/LConn1
  T_298873162__Itahue/LConn1 -- _CN_298873162_220000_CN_80518121_220000/LConn1
  T_298873162__Itahue/LConn2 -- _CN_298873162_220000_CN_80518121_220000/LConn2
  _CN_298873162_220000_CN_80518121_220000/LConn3 -- T_298873162__Itahue/LConn3 -- bus110/LConn1
  _CN_298873162_220000_CN_80518121_220000/RConn1 -- T_80518121__SE_Ancoa/LConn1 -- _CN_186477297_220000_CN_80518121_220000/LConn1
  _CN_298873162_220000_CN_80518121_220000/RConn2 -- T_80518121__SE_Ancoa/LConn2 -- _CN_186477297_220000_CN_80518121_220000/LConn2
  _CN_298873162_220000_CN_80518121_220000/RConn3 -- T_80518121__SE_Ancoa/LConn3 -- _CN_186477297_220000_CN_80518121_220000/LConn3 -- bus111/LConn1
  T_393463140__/LConn1 -- _CN_393463140_220000_CN_119834529_220000/RConn1
  T_393463140__/LConn2 -- _CN_393463140_220000_CN_119834529_220000/RConn2
  _CN_393463140_220000_CN_119834529_220000/RConn3 -- T_393463140__/LConn3 -- bus112/LConn1
  T_170066365__S_E_Gaby/LConn1 -- Línea_220_kV_El_Cobre_Gaby_57_km_189_MVA_CN_168852850_220000_CN_170066365_220000/RConn1
  T_170066365__S_E_Gaby/LConn2 -- Línea_220_kV_El_Cobre_Gaby_57_km_189_MVA_CN_168852850_220000_CN_170066365_220000/RConn2
  Línea_220_kV_El_Cobre_Gaby_57_km_189_MVA_CN_168852850_220000_CN_170066365_220000/RConn3 -- T_170066365__S_E_Gaby/LConn3 -- bus113/LConn1
  T_27215745__/LConn1 -- _CN_27215229_220000_CN_27215745_220000/RConn1
  T_27215745__/LConn2 -- _CN_27215229_220000_CN_27215745_220000/RConn2
  _CN_27215229_220000_CN_27215745_220000/RConn3 -- T_27215745__/LConn3 -- bus114/LConn1
  T_187680146__/LConn1 -- S_E_Charrúa___S_E_Coronel_1x220_kV_CN_187680146_220000_CN_167666088_220000/RConn1
  T_187680146__/LConn2 -- S_E_Charrúa___S_E_Coronel_1x220_kV_CN_187680146_220000_CN_167666088_220000/RConn2
  S_E_Charrúa___S_E_Coronel_1x220_kV_CN_187680146_220000_CN_167666088_220000/RConn3 -- T_187680146__/LConn3 -- bus115/LConn1
  T_98068896__/LConn1 -- _CN_98068896_220000_CN_139809239_220000/LConn1
  T_98068896__/LConn2 -- _CN_98068896_220000_CN_139809239_220000/LConn2
  _CN_98068896_220000_CN_139809239_220000/LConn3 -- T_98068896__/LConn3 -- bus116/LConn1
  T_139809239__/LConn1 -- _CN_98068896_220000_CN_139809239_220000/RConn1
  T_139809239__/LConn2 -- _CN_98068896_220000_CN_139809239_220000/RConn2
  _CN_98068896_220000_CN_139809239_220000/RConn3 -- T_139809239__/LConn3 -- bus117/LConn1
  T_186477297__/LConn1 -- _CN_186477297_220000_CN_80518121_220000/RConn1
  T_186477297__/LConn2 -- _CN_186477297_220000_CN_80518121_220000/RConn2
  _CN_186477297_220000_CN_80518121_220000/RConn3 -- T_186477297__/LConn3 -- bus118/LConn1
  T_167666093__Subestación_Charrúa_(Paño_500_kV)/LConn1 -- _CN_167666088_220000_CN_167666093_220000/RConn1
  T_167666093__Subestación_Charrúa_(Paño_500_kV)/LConn2 -- _CN_167666088_220000_CN_167666093_220000/RConn2
  _CN_167666088_220000_CN_167666093_220000/RConn3 -- T_167666093__Subestación_Charrúa_(Paño_500_kV)/LConn3 -- bus119/LConn1
  T_121436161__/RConn1 -- L_121436161/LConn1
  T_121436161__/RConn2 -- L_121436161/LConn2
  L_121436161/LConn3 -- T_121436161__/RConn3 -- bus120/LConn1
  T_119776135__/RConn1 -- L_119776135/LConn1
  T_119776135__/RConn2 -- L_119776135/LConn2
  L_119776135/LConn3 -- T_119776135__/RConn3 -- bus121/LConn1
  T_119889425__/RConn1 -- L_119889425/LConn1
  T_119889425__/RConn2 -- L_119889425/LConn2
  L_119889425/LConn3 -- T_119889425__/RConn3 -- bus122/LConn1
  T_30455625__SE_Los_Almendros/RConn1 -- L_30455625/LConn1
  T_30455625__SE_Los_Almendros/RConn2 -- L_30455625/LConn2
  L_30455625/LConn3 -- T_30455625__SE_Los_Almendros/RConn3 -- bus123/LConn1
  T_140087862__Subestacion_Eléctrica_San_Cristobal/RConn1 -- L_140087862/LConn1
  T_140087862__Subestacion_Eléctrica_San_Cristobal/RConn2 -- L_140087862/LConn2
  L_140087862/LConn3 -- T_140087862__Subestacion_Eléctrica_San_Cristobal/RConn3 -- bus124/LConn1
  T_321507700__/RConn1 -- L_321507700/LConn1
  T_321507700__/RConn2 -- L_321507700/LConn2
  L_321507700/LConn3 -- T_321507700__/RConn3 -- bus125/LConn1
  T_28321693__Subestación_San_Bernardo/RConn1 -- L_28321693/LConn1
  T_28321693__Subestación_San_Bernardo/RConn2 -- L_28321693/LConn2
  L_28321693/LConn3 -- T_28321693__Subestación_San_Bernardo/RConn3 -- bus126/LConn1
  T_28321441__/RConn1 -- L_28321441/LConn1
  T_28321441__/RConn2 -- L_28321441/LConn2
  L_28321441/LConn3 -- T_28321441__/RConn3 -- bus127/LConn1
  T_220292365__/RConn1 -- L_220292365/LConn1
  T_220292365__/RConn2 -- L_220292365/LConn2
  L_220292365/LConn3 -- T_220292365__/RConn3 -- bus128/LConn1
  T_394868441__/RConn1 -- L_394868441/LConn1
  T_394868441__/RConn2 -- L_394868441/LConn2
  L_394868441/LConn3 -- T_394868441__/RConn3 -- bus129/LConn1
  T_94811802__/RConn1 -- L_94811802/LConn1
  T_94811802__/RConn2 -- L_94811802/LConn2
  L_94811802/LConn3 -- T_94811802__/RConn3 -- bus130/LConn1
  T_236802012__/RConn1 -- L_236802012/LConn1
  T_236802012__/RConn2 -- L_236802012/LConn2
  L_236802012/LConn3 -- T_236802012__/RConn3 -- bus131/LConn1
  T_123910738__/RConn1 -- L_123910738/LConn1
  T_123910738__/RConn2 -- L_123910738/LConn2
  L_123910738/LConn3 -- T_123910738__/RConn3 -- bus132/LConn1
  T_205950704__/RConn1 -- L_205950704/LConn1
  T_205950704__/RConn2 -- L_205950704/LConn2
  L_205950704/LConn3 -- T_205950704__/RConn3 -- bus133/LConn1
  T_194041555__/RConn1 -- L_194041555/LConn1
  T_194041555__/RConn2 -- L_194041555/LConn2
  L_194041555/LConn3 -- T_194041555__/RConn3 -- bus134/LConn1
  T_94815220__/RConn1 -- L_94815220/LConn1
  T_94815220__/RConn2 -- L_94815220/LConn2
  L_94815220/LConn3 -- T_94815220__/RConn3 -- bus135/LConn1
  T_183356930__/RConn1 -- L_183356930/LConn1
  T_183356930__/RConn2 -- L_183356930/LConn2
  L_183356930/LConn3 -- T_183356930__/RConn3 -- bus136/LConn1
  T_182692487__/RConn1 -- L_182692487/LConn1
  T_182692487__/RConn2 -- L_182692487/LConn2
  L_182692487/LConn3 -- T_182692487__/RConn3 -- bus137/LConn1
  T_169337349__S_E_Angamos___Eléctrica_Angamos/RConn1 -- L_169337349/LConn1
  T_169337349__S_E_Angamos___Eléctrica_Angamos/RConn2 -- L_169337349/LConn2
  L_169337349/LConn3 -- T_169337349__S_E_Angamos___Eléctrica_Angamos/RConn3 -- bus138/LConn1
  T_168851504__/RConn1 -- L_168851504/LConn1
  T_168851504__/RConn2 -- L_168851504/LConn2
  L_168851504/LConn3 -- T_168851504__/RConn3 -- bus139/LConn1
  T_157553674__Subestacion_Pozo_Almonte/RConn1 -- L_157553674/LConn1
  T_157553674__Subestacion_Pozo_Almonte/RConn2 -- L_157553674/LConn2
  L_157553674/LConn3 -- T_157553674__Subestacion_Pozo_Almonte/RConn3 -- bus140/LConn1
  T_182735456__S_E_Lagunas/RConn1 -- L_182735456/LConn1
  T_182735456__S_E_Lagunas/RConn2 -- L_182735456/LConn2
  L_182735456/LConn3 -- T_182735456__S_E_Lagunas/RConn3 -- bus141/LConn1
  T_394165771__/RConn1 -- L_394165771/LConn1
  T_394165771__/RConn2 -- L_394165771/LConn2
  L_394165771/LConn3 -- T_394165771__/RConn3 -- bus142/LConn1
  T_349891827__S_E_Polpaico/RConn1 -- L_349891827/LConn1
  T_349891827__S_E_Polpaico/RConn2 -- L_349891827/LConn2
  L_349891827/LConn3 -- T_349891827__S_E_Polpaico/RConn3 -- bus143/LConn1
  T_236594201__/RConn1 -- L_236594201/LConn1
  T_236594201__/RConn2 -- L_236594201/LConn2
  L_236594201/LConn3 -- T_236594201__/RConn3 -- bus144/LConn1
  T_121431104__Domeyko/RConn1 -- L_121431104/LConn1
  T_121431104__Domeyko/RConn2 -- L_121431104/LConn2
  L_121431104/LConn3 -- T_121431104__Domeyko/RConn3 -- bus145/LConn1
  T_182235178__/RConn1 -- L_182235178/LConn1
  T_182235178__/RConn2 -- L_182235178/LConn2
  L_182235178/LConn3 -- T_182235178__/RConn3 -- bus146/LConn1
  T_119834529__Cardones/RConn1 -- L_119834529/LConn1
  T_119834529__Cardones/RConn2 -- L_119834529/LConn2
  L_119834529/LConn3 -- T_119834529__Cardones/RConn3 -- bus147/LConn1
  T_182236045__/RConn1 -- L_182236045/LConn1
  T_182236045__/RConn2 -- L_182236045/LConn2
  L_182236045/LConn3 -- T_182236045__/RConn3 -- bus148/LConn1
  T_118304300__/RConn1 -- L_118304300/LConn1
  T_118304300__/RConn2 -- L_118304300/LConn2
  L_118304300/LConn3 -- T_118304300__/RConn3 -- bus149/LConn1
  T_167666088__Subestación_Charrúa_(Paño_220_kV)/RConn1 -- L_167666088/LConn1
  T_167666088__Subestación_Charrúa_(Paño_220_kV)/RConn2 -- L_167666088/LConn2
  L_167666088/LConn3 -- T_167666088__Subestación_Charrúa_(Paño_220_kV)/RConn3 -- bus150/LConn1
  T_395644253__/RConn1 -- L_395644253/LConn1
  T_395644253__/RConn2 -- L_395644253/LConn2
  L_395644253/LConn3 -- T_395644253__/RConn3 -- bus151/LConn1
  T_140002904__Temuco/RConn1 -- L_140002904/LConn1
  T_140002904__Temuco/RConn2 -- L_140002904/LConn2
  L_140002904/LConn3 -- T_140002904__Temuco/RConn3 -- bus152/LConn1
  T_120102647__/RConn1 -- L_120102647/LConn1
  T_120102647__/RConn2 -- L_120102647/LConn2
  L_120102647/LConn3 -- T_120102647__/RConn3 -- bus153/LConn1
  T_187100722__S_E_Cautín/RConn1 -- L_187100722/LConn1
  T_187100722__S_E_Cautín/RConn2 -- L_187100722/LConn2
  L_187100722/LConn3 -- T_187100722__S_E_Cautín/RConn3 -- bus154/LConn1
  T_190325675__/RConn1 -- L_190325675/LConn1
  T_190325675__/RConn2 -- L_190325675/LConn2
  L_190325675/LConn3 -- T_190325675__/RConn3 -- bus155/LConn1
  T_182803372__Valdivia/RConn1 -- L_182803372/LConn1
  T_182803372__Valdivia/RConn2 -- L_182803372/LConn2
  L_182803372/LConn3 -- T_182803372__Valdivia/RConn3 -- bus156/LConn1
  T_354354025__S_E_Mulchén/RConn1 -- L_354354025/LConn1
  T_354354025__S_E_Mulchén/RConn2 -- L_354354025/LConn2
  L_354354025/LConn3 -- T_354354025__S_E_Mulchén/RConn3 -- bus157/LConn1
  T_121431094__/RConn1 -- L_121431094/LConn1
  T_121431094__/RConn2 -- L_121431094/LConn2
  L_121431094/LConn3 -- T_121431094__/RConn3 -- bus158/LConn1
  T_30641904_110000_S_E_O'higgins/RConn1 -- L_30641904/LConn1
  T_30641904_110000_S_E_O'higgins/RConn2 -- L_30641904/LConn2
  L_30641904/LConn3 -- T_30641904_110000_S_E_O'higgins/RConn3 -- bus159/LConn1
  T_121236949__/RConn1 -- L_121236949/LConn1
  T_121236949__/RConn2 -- L_121236949/LConn2
  L_121236949/LConn3 -- T_121236949__/RConn3 -- bus160/LConn1
  T_200239163__/RConn1 -- L_200239163/LConn1
  T_200239163__/RConn2 -- L_200239163/LConn2
  L_200239163/LConn3 -- T_200239163__/RConn3 -- bus161/LConn1
  T_200067463__/RConn1 -- L_200067463/LConn1
  T_200067463__/RConn2 -- L_200067463/LConn2
  L_200067463/LConn3 -- T_200067463__/RConn3 -- bus162/LConn1
  T_121455793__Lagunas_Seca/RConn1 -- L_121455793/LConn1
  T_121455793__Lagunas_Seca/RConn2 -- L_121455793/LConn2
  L_121455793/LConn3 -- T_121455793__Lagunas_Seca/RConn3 -- bus163/LConn1
  T_328656452__S_E_Mantos_Blancos/RConn1 -- L_328656452/LConn1
  T_328656452__S_E_Mantos_Blancos/RConn2 -- L_328656452/LConn2
  L_328656452/LConn3 -- T_328656452__S_E_Mantos_Blancos/RConn3 -- bus164/LConn1
  T_30641628__S_E_Chacaya/RConn1 -- L_30641628/LConn1
  T_30641628__S_E_Chacaya/RConn2 -- L_30641628/LConn2
  L_30641628/LConn3 -- T_30641628__S_E_Chacaya/RConn3 -- bus165/LConn1
  T_120712016__S_E_Capricornio/RConn1 -- L_120712016/LConn1
  T_120712016__S_E_Capricornio/RConn2 -- L_120712016/LConn2
  L_120712016/LConn3 -- T_120712016__S_E_Capricornio/RConn3 -- bus166/LConn1
  T_121623737__Laberinto/RConn1 -- L_121623737/LConn1
  T_121623737__Laberinto/RConn2 -- L_121623737/LConn2
  L_121623737/LConn3 -- T_121623737__Laberinto/RConn3 -- bus167/LConn1
  T_145413703__/RConn1 -- L_145413703/LConn1
  T_145413703__/RConn2 -- L_145413703/LConn2
  L_145413703/LConn3 -- T_145413703__/RConn3 -- bus168/LConn1
  T_24411638__Sub_Estacion_Melipulli/RConn1 -- L_24411638/LConn1
  T_24411638__Sub_Estacion_Melipulli/RConn2 -- L_24411638/LConn2
  L_24411638/LConn3 -- T_24411638__Sub_Estacion_Melipulli/RConn3 -- bus169/LConn1
  T_170017864__S_E_El_Abra/RConn1 -- L_170017864/LConn1
  T_170017864__S_E_El_Abra/RConn2 -- L_170017864/LConn2
  L_170017864/LConn3 -- T_170017864__S_E_El_Abra/RConn3 -- bus170/LConn1
  T_111486352__S_E_Crucero/RConn1 -- L_111486352/LConn1
  T_111486352__S_E_Crucero/RConn2 -- L_111486352/LConn2
  L_111486352/LConn3 -- T_111486352__S_E_Crucero/RConn3 -- bus171/LConn1
  T_328652522__S_E_Rodomiro_Tomic/RConn1 -- L_328652522/LConn1
  T_328652522__S_E_Rodomiro_Tomic/RConn2 -- L_328652522/LConn2
  L_328652522/LConn3 -- T_328652522__S_E_Rodomiro_Tomic/RConn3 -- bus172/LConn1
  T_121454923__Nueva_Zaldivar/RConn1 -- L_121454923/LConn1
  T_121454923__Nueva_Zaldivar/RConn2 -- L_121454923/LConn2
  L_121454923/LConn3 -- T_121454923__Nueva_Zaldivar/RConn3 -- bus173/LConn1
  T_121445157__P__Óxidos/RConn1 -- L_121445157/LConn1
  T_121445157__P__Óxidos/RConn2 -- L_121445157/LConn2
  L_121445157/LConn3 -- T_121445157__P__Óxidos/RConn3 -- bus174/LConn1
  T_321511794__Zaldivar/RConn1 -- L_321511794/LConn1
  T_321511794__Zaldivar/RConn2 -- L_321511794/LConn2
  L_321511794/LConn3 -- T_321511794__Zaldivar/RConn3 -- bus175/LConn1
  T_321520065__Lomas_Bayas/RConn1 -- L_321520065/LConn1
  T_321520065__Lomas_Bayas/RConn2 -- L_321520065/LConn2
  L_321520065/LConn3 -- T_321520065__Lomas_Bayas/RConn3 -- bus176/LConn1
  T_168852850__S_E_El_Cobre/RConn1 -- L_168852850/LConn1
  T_168852850__S_E_El_Cobre/RConn2 -- L_168852850/LConn2
  L_168852850/LConn3 -- T_168852850__S_E_El_Cobre/RConn3 -- bus177/LConn1
  T_136149844__Abengoa/RConn1 -- L_136149844/LConn1
  T_136149844__Abengoa/RConn2 -- L_136149844/LConn2
  L_136149844/LConn3 -- T_136149844__Abengoa/RConn3 -- bus178/LConn1
  T_170073895__Oeste/RConn1 -- L_170073895/LConn1
  T_170073895__Oeste/RConn2 -- L_170073895/LConn2
  L_170073895/LConn3 -- T_170073895__Oeste/RConn3 -- bus179/LConn1
  T_182692483__/RConn1 -- L_182692483/LConn1
  T_182692483__/RConn2 -- L_182692483/LConn2
  L_182692483/LConn3 -- T_182692483__/RConn3 -- bus180/LConn1
  T_187201126__/RConn1 -- L_187201126/LConn1
  T_187201126__/RConn2 -- L_187201126/LConn2
  L_187201126/LConn3 -- T_187201126__/RConn3 -- bus181/LConn1
  T_375149685__/RConn1 -- L_375149685/LConn1
  T_375149685__/RConn2 -- L_375149685/LConn2
  L_375149685/LConn3 -- T_375149685__/RConn3 -- bus182/LConn1
  T_393489602__/RConn1 -- L_393489602/LConn1
  T_393489602__/RConn2 -- L_393489602/LConn2
  L_393489602/LConn3 -- T_393489602__/RConn3 -- bus183/LConn1
  T_170022524__El_Tesoro/RConn1 -- L_170022524/LConn1
  T_170022524__El_Tesoro/RConn2 -- L_170022524/LConn2
  L_170022524/LConn3 -- T_170022524__El_Tesoro/RConn3 -- bus184/LConn1
  T_170022526__Esperanza/RConn1 -- L_170022526/LConn1
  T_170022526__Esperanza/RConn2 -- L_170022526/LConn2
  L_170022526/LConn3 -- T_170022526__Esperanza/RConn3 -- bus185/LConn1
  T_111486348__S_E_Encuentro/RConn1 -- L_111486348/LConn1
  T_111486348__S_E_Encuentro/RConn2 -- L_111486348/LConn2
  L_111486348/LConn3 -- T_111486348__S_E_Encuentro/RConn3 -- bus186/LConn1
  T_182747576__S_E_Quebrada_blanca/RConn1 -- L_182747576/LConn1
  T_182747576__S_E_Quebrada_blanca/RConn2 -- L_182747576/LConn2
  L_182747576/LConn3 -- T_182747576__S_E_Quebrada_blanca/RConn3 -- bus187/LConn1
  T_226755205_220000_Paposo/RConn1 -- L_226755205/LConn1
  T_226755205_220000_Paposo/RConn2 -- L_226755205/LConn2
  L_226755205/LConn3 -- T_226755205_220000_Paposo/RConn3 -- bus188/LConn1
  T_219477643__Central_Canela_II/RConn1 -- L_219477643/LConn1
  T_219477643__Central_Canela_II/RConn2 -- L_219477643/LConn2
  L_219477643/LConn3 -- T_219477643__Central_Canela_II/RConn3 -- bus189/LConn1
  T_119688342__Carrera_Pinto/RConn1 -- L_119688342/LConn1
  T_119688342__Carrera_Pinto/RConn2 -- L_119688342/LConn2
  L_119688342/LConn3 -- T_119688342__Carrera_Pinto/RConn3 -- bus190/LConn1
  T_253852513__/RConn1 -- L_253852513/LConn1
  T_253852513__/RConn2 -- L_253852513/LConn2
  L_253852513/LConn3 -- T_253852513__/RConn3 -- bus191/LConn1
  T_140162733__/RConn1 -- L_140162733/LConn1
  T_140162733__/RConn2 -- L_140162733/LConn2
  L_140162733/LConn3 -- T_140162733__/RConn3 -- bus192/LConn1
  T_170023614__/RConn1 -- L_170023614/LConn1
  T_170023614__/RConn2 -- L_170023614/LConn2
  L_170023614/LConn3 -- T_170023614__/RConn3 -- bus193/LConn1
  T_393489604__/RConn1 -- L_393489604/LConn1
  T_393489604__/RConn2 -- L_393489604/LConn2
  L_393489604/LConn3 -- T_393489604__/RConn3 -- bus194/LConn1
  T_120860874__S_E_Atacama/RConn1 -- L_120860874/LConn1
  T_120860874__S_E_Atacama/RConn2 -- L_120860874/LConn2
  L_120860874/LConn3 -- T_120860874__S_E_Atacama/RConn3 -- bus195/LConn1
  T_120707837__/RConn1 -- L_120707837/LConn1
  T_120707837__/RConn2 -- L_120707837/LConn2
  L_120707837/LConn3 -- T_120707837__/RConn3 -- bus196/LConn1
  T_120960385__S_E_Mejillones/RConn1 -- L_120960385/LConn1
  T_120960385__S_E_Mejillones/RConn2 -- L_120960385/LConn2
  L_120960385/LConn3 -- T_120960385__S_E_Mejillones/RConn3 -- bus197/LConn1
  T_88147668__/RConn1 -- L_88147668/LConn1
  T_88147668__/RConn2 -- L_88147668/LConn2
  L_88147668/LConn3 -- T_88147668__/RConn3 -- bus198/LConn1
  T_110804340__S_E_Condores/RConn1 -- L_110804340/LConn1
  T_110804340__S_E_Condores/RConn2 -- L_110804340/LConn2
  L_110804340/LConn3 -- T_110804340__S_E_Condores/RConn3 -- bus199/LConn1
  T_180536025__/RConn1 -- L_180536025/LConn1
  T_180536025__/RConn2 -- L_180536025/LConn2
  L_180536025/LConn3 -- T_180536025__/RConn3 -- bus200/LConn1
  T_120471866__Coloso_220_kV/RConn1 -- L_120471866/LConn1
  T_120471866__Coloso_220_kV/RConn2 -- L_120471866/LConn2
  L_120471866/LConn3 -- T_120471866__Coloso_220_kV/RConn3 -- bus201/LConn1
  T_184191729__/RConn1 -- L_184191729/LConn1
  T_184191729__/RConn2 -- L_184191729/LConn2
  L_184191729/LConn3 -- T_184191729__/RConn3 -- bus202/LConn1
  T_184197597__/RConn1 -- L_184197597/LConn1
  T_184197597__/RConn2 -- L_184197597/LConn2
  L_184197597/LConn3 -- T_184197597__/RConn3 -- bus203/LConn1
  T_349891826__S_E_Polpaico/RConn1 -- L_349891826/LConn1
  T_349891826__S_E_Polpaico/RConn2 -- L_349891826/LConn2
  L_349891826/LConn3 -- T_349891826__S_E_Polpaico/RConn3 -- bus204/LConn1
  T_27215229__/RConn1 -- L_27215229/LConn1
  T_27215229__/RConn2 -- L_27215229/LConn2
  L_27215229/LConn3 -- T_27215229__/RConn3 -- bus205/LConn1
  T_123909946__/RConn1 -- L_123909946/LConn1
  T_123909946__/RConn2 -- L_123909946/LConn2
  L_123909946/LConn3 -- T_123909946__/RConn3 -- bus206/LConn1
  T_155008260__/RConn1 -- L_155008260/LConn1
  T_155008260__/RConn2 -- L_155008260/LConn2
  L_155008260/LConn3 -- T_155008260__/RConn3 -- bus207/LConn1
  T_91655961_220000_Subestacion_Electrica_Los_Vilos/RConn1 -- L_91655961/LConn1
  T_91655961_220000_Subestacion_Electrica_Los_Vilos/RConn2 -- L_91655961/LConn2
  L_91655961/LConn3 -- T_91655961_220000_Subestacion_Electrica_Los_Vilos/RConn3 -- bus208/LConn1
  T_120791316__S_E_Esmeralda/RConn1 -- L_120791316/LConn1
  T_120791316__S_E_Esmeralda/RConn2 -- L_120791316/LConn2
  L_120791316/LConn3 -- T_120791316__S_E_Esmeralda/RConn3 -- bus209/LConn1
  T_120791326__S_E_Esmeralda_Centro/RConn1 -- L_120791326/LConn1
  T_120791326__S_E_Esmeralda_Centro/RConn2 -- L_120791326/LConn2
  L_120791326/LConn3 -- T_120791326__S_E_Esmeralda_Centro/RConn3 -- bus210/LConn1
  T_110801625__Tarapacá/RConn1 -- L_110801625/LConn1
  T_110801625__Tarapacá/RConn2 -- L_110801625/LConn2
  L_110801625/LConn3 -- T_110801625__Tarapacá/RConn3 -- bus211/LConn1
  T_168492929__/RConn1 -- L_168492929/LConn1
  T_168492929__/RConn2 -- L_168492929/LConn2
  L_168492929/LConn3 -- T_168492929__/RConn3 -- bus212/LConn1
  T_298873162__Itahue/RConn1 -- L_298873162/LConn1
  T_298873162__Itahue/RConn2 -- L_298873162/LConn2
  L_298873162/LConn3 -- T_298873162__Itahue/RConn3 -- bus213/LConn1
  T_80518121__SE_Ancoa/RConn1 -- L_80518121/LConn1
  T_80518121__SE_Ancoa/RConn2 -- L_80518121/LConn2
  L_80518121/LConn3 -- T_80518121__SE_Ancoa/RConn3 -- bus214/LConn1
  T_393463140__/RConn1 -- L_393463140/LConn1
  T_393463140__/RConn2 -- L_393463140/LConn2
  L_393463140/LConn3 -- T_393463140__/RConn3 -- bus215/LConn1
  T_170066365__S_E_Gaby/RConn1 -- L_170066365/LConn1
  T_170066365__S_E_Gaby/RConn2 -- L_170066365/LConn2
  L_170066365/LConn3 -- T_170066365__S_E_Gaby/RConn3 -- bus216/LConn1
  T_27215745__/RConn1 -- L_27215745/LConn1
  T_27215745__/RConn2 -- L_27215745/LConn2
  L_27215745/LConn3 -- T_27215745__/RConn3 -- bus217/LConn1
  T_187680146__/RConn1 -- L_187680146/LConn1
  T_187680146__/RConn2 -- L_187680146/LConn2
  L_187680146/LConn3 -- T_187680146__/RConn3 -- bus218/LConn1
  T_98068896__/RConn1 -- L_98068896/LConn1
  T_98068896__/RConn2 -- L_98068896/LConn2
  L_98068896/LConn3 -- T_98068896__/RConn3 -- bus219/LConn1
  T_139809239__/RConn1 -- L_139809239/LConn1
  T_139809239__/RConn2 -- L_139809239/LConn2
  L_139809239/LConn3 -- T_139809239__/RConn3 -- bus220/LConn1
  T_186477297__/RConn1 -- L_186477297/LConn1
  T_186477297__/RConn2 -- L_186477297/LConn2
  L_186477297/LConn3 -- T_186477297__/RConn3 -- bus221/LConn1
  T_167666093__Subestación_Charrúa_(Paño_500_kV)/RConn1 -- L_167666093/LConn1
  T_167666093__Subestación_Charrúa_(Paño_500_kV)/RConn2 -- L_167666093/LConn2
  L_167666093/LConn3 -- T_167666093__Subestación_Charrúa_(Paño_500_kV)/RConn3 -- bus222/LConn1
